simulink model "pfb_fir_1024c_32i_core"  (R2019a)
(part 4 of 32)

      |     set_param(gcb, 'MaskVisibilities',{'on','on','on','on','on'});
      | end
  pol1_in6_tap2 : Subsystem  AncestorBlock=casper_library_pfbs/tap_real  mask(pfb_tap_real){mult_latency=2, coeff_width=18, coeff_frac_width=17, delay=64, data_width=8, bram_latency=2, use_hdl=on, use_embedded=off}
      mask prompts: mult_latency "Multiplier Latency"; coeff_width "Coefficient Bit Width In"; coeff_frac_width "Coefficient Fractional Bits"; delay "Data/Sync Delay"; data_width "Data Bit Width In"; bram_latency "BRAM Latency"; use_hdl "Use behavioral HDL for multlipliers"; use_embedded "Use embedded multipliers"
      mask init: same as pfb_fir_1024c_32i_core/pfb_fir_real/pol1_in10_tap2
  pol1_in6_tap3 : Subsystem  AncestorBlock=casper_library_pfbs/tap_real  mask(pfb_tap_real){mult_latency=2, coeff_width=18, coeff_frac_width=17, delay=64, data_width=8, bram_latency=2, use_hdl=on, use_embedded=off}
      mask prompts: mult_latency "Multiplier Latency"; coeff_width "Coefficient Bit Width In"; coeff_frac_width "Coefficient Fractional Bits"; delay "Data/Sync Delay"; data_width "Data Bit Width In"; bram_latency "BRAM Latency"; use_hdl "Use behavioral HDL for multlipliers"; use_embedded "Use embedded multipliers"
      mask init: same as pfb_fir_1024c_32i_core/pfb_fir_real/pol1_in10_tap2
  pol1_in6_tap4 : Subsystem  AncestorBlock=casper_library_pfbs/tap_real  mask(pfb_tap_real){mult_latency=2, coeff_width=18, coeff_frac_width=17, delay=64, data_width=8, bram_latency=2, use_hdl=on, use_embedded=off}
      mask prompts: mult_latency "Multiplier Latency"; coeff_width "Coefficient Bit Width In"; coeff_frac_width "Coefficient Fractional Bits"; delay "Data/Sync Delay"; data_width "Data Bit Width In"; bram_latency "BRAM Latency"; use_hdl "Use behavioral HDL for multlipliers"; use_embedded "Use embedded multipliers"
      mask init: same as pfb_fir_1024c_32i_core/pfb_fir_real/pol1_in10_tap2
  pol1_in6_tap5 : Subsystem  AncestorBlock=casper_library_pfbs/tap_real  mask(pfb_tap_real){mult_latency=2, coeff_width=18, coeff_frac_width=17, delay=64, data_width=8, bram_latency=2, use_hdl=on, use_embedded=off}
      mask prompts: mult_latency "Multiplier Latency"; coeff_width "Coefficient Bit Width In"; coeff_frac_width "Coefficient Fractional Bits"; delay "Data/Sync Delay"; data_width "Data Bit Width In"; bram_latency "BRAM Latency"; use_hdl "Use behavioral HDL for multlipliers"; use_embedded "Use embedded multipliers"
      mask init: same as pfb_fir_1024c_32i_core/pfb_fir_real/pol1_in10_tap2
  pol1_in6_tap6 : Subsystem  AncestorBlock=casper_library_pfbs/tap_real  mask(pfb_tap_real){mult_latency=2, coeff_width=18, coeff_frac_width=17, delay=64, data_width=8, bram_latency=2, use_hdl=on, use_embedded=off}
      mask prompts: mult_latency "Multiplier Latency"; coeff_width "Coefficient Bit Width In"; coeff_frac_width "Coefficient Fractional Bits"; delay "Data/Sync Delay"; data_width "Data Bit Width In"; bram_latency "BRAM Latency"; use_hdl "Use behavioral HDL for multlipliers"; use_embedded "Use embedded multipliers"
      mask init: same as pfb_fir_1024c_32i_core/pfb_fir_real/pol1_in10_tap2
  pol1_in6_tap7 : Subsystem  AncestorBlock=casper_library_pfbs/tap_real  mask(pfb_tap_real){mult_latency=2, coeff_width=18, coeff_frac_width=17, delay=64, data_width=8, bram_latency=2, use_hdl=on, use_embedded=off}
      mask prompts: mult_latency "Multiplier Latency"; coeff_width "Coefficient Bit Width In"; coeff_frac_width "Coefficient Fractional Bits"; delay "Data/Sync Delay"; data_width "Data Bit Width In"; bram_latency "BRAM Latency"; use_hdl "Use behavioral HDL for multlipliers"; use_embedded "Use embedded multipliers"
      mask init: same as pfb_fir_1024c_32i_core/pfb_fir_real/pol1_in10_tap2
  pol1_in7_coeffs : Subsystem  AncestorBlock=casper_library_pfbs/pfb_coeff_gen  mask(pfb_coeff_gen){PFBSize=11, CoeffBitWidth=18, TotalTaps=8, CoeffDistMem=off, WindowType=hamming, bram_latency=2, n_inputs=5, nput=6, fwidth=1, debug_mode=off, fan_latency=1}
      mask prompts: PFBSize "Size of PFB: (2^? pnts)"; CoeffBitWidth "Bitwidth of Coefficients:"; TotalTaps "Total Number of Taps:"; CoeffDistMem "Implement Coeff Gen in Distributed Memory"; WindowType "Windowing Function:"; bram_latency "BRAM Latency"; n_inputs "Number of Simultaneous Inputs: (2^?)"; nput "This is input number:"; fwidth "Bin Width (normal=1)"; debug_mode "Debug mode - coeffs are a [1:pfb_size*taps] ramp."; fan_latency "Fanout latency"
      mask init: same as pfb_fir_1024c_32i_core/pfb_fir_real/pol1_in10_coeffs
      settings: AttributesFormatString=|
      | PFBSize=11, n_inputs=5,
      | taps=8, input=6
  pol1_in7_first_tap : Subsystem  AncestorBlock=casper_library_pfbs/first_tap_real  mask(first_tap_real){PFBSize=11, CoeffBitWidth=18, TotalTaps=8, BitWidthIn=8, WindowType=hamming, mult_latency=2, bram_latency=2, n_inputs=5, fwidth=1, use_hdl=on, use_embedded=off}
      mask prompts: PFBSize "Size of PFB: (2^? pnts)"; CoeffBitWidth "Bitwidth of Coefficients:"; TotalTaps "Total Number of Taps:"; BitWidthIn "Input Bitwidth:"; WindowType "Windowing Function:"; mult_latency "Mult Latency"; bram_latency "BRAM Latency"; n_inputs "Number of Simultaneous Inputs: (2^?)"; fwidth "Bit Width (normal=1)"; use_hdl "Use behavioral HDL for multlipliers"; use_embedded "Use embedded multipliers"
      mask init: same as pfb_fir_1024c_32i_core/pfb_fir_real/pol1_in10_first_tap
      settings: AttributesFormatString=taps=8
      mask TypeOptions WindowType: bartlett | barthannwin | blackman | blackmanharris | bohamwin | chebwin | flattopwin | gausswin | hamming | hann | kaiser | nuttallwin | parzenwin | rectwin | tukeywin | triang | userwindow
      mask Callback use_hdl:
      | use_hdl = get_param(gcb,'use_hdl');
      | if( strcmp(use_hdl,'on')),
      |     set_param(gcb, 'use_embedded','off');
      |     set_param(gcb, 'MaskVisibilities',{'on','on','on','on','on','on','on','on','on','on','off'});
      | else,
      |     set_param(gcb, 'MaskVisibilities',{'on','on','on','on','on','on','on','on','on','on','on'});
      | end
  pol1_in7_last_tap : Subsystem  AncestorBlock=casper_library_pfbs/last_tap_real  mask(last_tap_real){BitWidthIn=8, CoeffBitWidth=18, mult_latency=2, use_hdl=on, use_embedded=off}
      mask prompts: BitWidthIn "Input Bitwidth:"; CoeffBitWidth "Coeff Bitwidth:"; mult_latency "Mult Latency"; use_hdl "Use behavioral HDL for multlipliers"; use_embedded "Use embedded multipliers"
      mask init:
      | last_tap_real_init(gcb,...
      |     'BitWidthIn', BitWidthIn,...
      |     'CoeffBitWidth', CoeffBitWidth,...
      |     'mult_latency', mult_latency,...
      |     'use_hdl', use_hdl,...
      |     'use_embedded', use_embedded);
      mask Callback use_hdl:
      | use_hdl = get_param(gcb,'use_hdl');
      | if( strcmp(use_hdl,'on')),
      |     set_param(gcb, 'use_embedded','off');
      |     set_param(gcb, 'MaskVisibilities',{'on','on','on','on','off'});
      | else,
      |     set_param(gcb, 'MaskVisibilities',{'on','on','on','on','on'});
      | end
  pol1_in7_tap2 : Subsystem  AncestorBlock=casper_library_pfbs/tap_real  mask(pfb_tap_real){mult_latency=2, coeff_width=18, coeff_frac_width=17, delay=64, data_width=8, bram_latency=2, use_hdl=on, use_embedded=off}
      mask prompts: mult_latency "Multiplier Latency"; coeff_width "Coefficient Bit Width In"; coeff_frac_width "Coefficient Fractional Bits"; delay "Data/Sync Delay"; data_width "Data Bit Width In"; bram_latency "BRAM Latency"; use_hdl "Use behavioral HDL for multlipliers"; use_embedded "Use embedded multipliers"
      mask init: same as pfb_fir_1024c_32i_core/pfb_fir_real/pol1_in10_tap2
  pol1_in7_tap3 : Subsystem  AncestorBlock=casper_library_pfbs/tap_real  mask(pfb_tap_real){mult_latency=2, coeff_width=18, coeff_frac_width=17, delay=64, data_width=8, bram_latency=2, use_hdl=on, use_embedded=off}
      mask prompts: mult_latency "Multiplier Latency"; coeff_width "Coefficient Bit Width In"; coeff_frac_width "Coefficient Fractional Bits"; delay "Data/Sync Delay"; data_width "Data Bit Width In"; bram_latency "BRAM Latency"; use_hdl "Use behavioral HDL for multlipliers"; use_embedded "Use embedded multipliers"
      mask init: same as pfb_fir_1024c_32i_core/pfb_fir_real/pol1_in10_tap2
  pol1_in7_tap4 : Subsystem  AncestorBlock=casper_library_pfbs/tap_real  mask(pfb_tap_real){mult_latency=2, coeff_width=18, coeff_frac_width=17, delay=64, data_width=8, bram_latency=2, use_hdl=on, use_embedded=off}
      mask prompts: mult_latency "Multiplier Latency"; coeff_width "Coefficient Bit Width In"; coeff_frac_width "Coefficient Fractional Bits"; delay "Data/Sync Delay"; data_width "Data Bit Width In"; bram_latency "BRAM Latency"; use_hdl "Use behavioral HDL for multlipliers"; use_embedded "Use embedded multipliers"
      mask init: same as pfb_fir_1024c_32i_core/pfb_fir_real/pol1_in10_tap2
  pol1_in7_tap5 : Subsystem  AncestorBlock=casper_library_pfbs/tap_real  mask(pfb_tap_real){mult_latency=2, coeff_width=18, coeff_frac_width=17, delay=64, data_width=8, bram_latency=2, use_hdl=on, use_embedded=off}
      mask prompts: mult_latency "Multiplier Latency"; coeff_width "Coefficient Bit Width In"; coeff_frac_width "Coefficient Fractional Bits"; delay "Data/Sync Delay"; data_width "Data Bit Width In"; bram_latency "BRAM Latency"; use_hdl "Use behavioral HDL for multlipliers"; use_embedded "Use embedded multipliers"
      mask init: same as pfb_fir_1024c_32i_core/pfb_fir_real/pol1_in10_tap2
  pol1_in7_tap6 : Subsystem  AncestorBlock=casper_library_pfbs/tap_real  mask(pfb_tap_real){mult_latency=2, coeff_width=18, coeff_frac_width=17, delay=64, data_width=8, bram_latency=2, use_hdl=on, use_embedded=off}
      mask prompts: mult_latency "Multiplier Latency"; coeff_width "Coefficient Bit Width In"; coeff_frac_width "Coefficient Fractional Bits"; delay "Data/Sync Delay"; data_width "Data Bit Width In"; bram_latency "BRAM Latency"; use_hdl "Use behavioral HDL for multlipliers"; use_embedded "Use embedded multipliers"
      mask init: same as pfb_fir_1024c_32i_core/pfb_fir_real/pol1_in10_tap2
  pol1_in7_tap7 : Subsystem  AncestorBlock=casper_library_pfbs/tap_real  mask(pfb_tap_real){mult_latency=2, coeff_width=18, coeff_frac_width=17, delay=64, data_width=8, bram_latency=2, use_hdl=on, use_embedded=off}
      mask prompts: mult_latency "Multiplier Latency"; coeff_width "Coefficient Bit Width In"; coeff_frac_width "Coefficient Fractional Bits"; delay "Data/Sync Delay"; data_width "Data Bit Width In"; bram_latency "BRAM Latency"; use_hdl "Use behavioral HDL for multlipliers"; use_embedded "Use embedded multipliers"
      mask init: same as pfb_fir_1024c_32i_core/pfb_fir_real/pol1_in10_tap2
  pol1_in8_coeffs : Subsystem  AncestorBlock=casper_library_pfbs/pfb_coeff_gen  mask(pfb_coeff_gen){PFBSize=11, CoeffBitWidth=18, TotalTaps=8, CoeffDistMem=off, WindowType=hamming, bram_latency=2, n_inputs=5, nput=7, fwidth=1, debug_mode=off, fan_latency=1}
      mask prompts: PFBSize "Size of PFB: (2^? pnts)"; CoeffBitWidth "Bitwidth of Coefficients:"; TotalTaps "Total Number of Taps:"; CoeffDistMem "Implement Coeff Gen in Distributed Memory"; WindowType "Windowing Function:"; bram_latency "BRAM Latency"; n_inputs "Number of Simultaneous Inputs: (2^?)"; nput "This is input number:"; fwidth "Bin Width (normal=1)"; debug_mode "Debug mode - coeffs are a [1:pfb_size*taps] ramp."; fan_latency "Fanout latency"
      mask init: same as pfb_fir_1024c_32i_core/pfb_fir_real/pol1_in10_coeffs
      settings: AttributesFormatString=|
      | PFBSize=11, n_inputs=5,
      | taps=8, input=7
  pol1_in8_first_tap : Subsystem  AncestorBlock=casper_library_pfbs/first_tap_real  mask(first_tap_real){PFBSize=11, CoeffBitWidth=18, TotalTaps=8, BitWidthIn=8, WindowType=hamming, mult_latency=2, bram_latency=2, n_inputs=5, fwidth=1, use_hdl=on, use_embedded=off}
      mask prompts: PFBSize "Size of PFB: (2^? pnts)"; CoeffBitWidth "Bitwidth of Coefficients:"; TotalTaps "Total Number of Taps:"; BitWidthIn "Input Bitwidth:"; WindowType "Windowing Function:"; mult_latency "Mult Latency"; bram_latency "BRAM Latency"; n_inputs "Number of Simultaneous Inputs: (2^?)"; fwidth "Bit Width (normal=1)"; use_hdl "Use behavioral HDL for multlipliers"; use_embedded "Use embedded multipliers"
      mask init: same as pfb_fir_1024c_32i_core/pfb_fir_real/pol1_in10_first_tap
      settings: AttributesFormatString=taps=8
      mask TypeOptions WindowType: bartlett | barthannwin | blackman | blackmanharris | bohamwin | chebwin | flattopwin | gausswin | hamming | hann | kaiser | nuttallwin | parzenwin | rectwin | tukeywin | triang | userwindow
      mask Callback use_hdl:
      | use_hdl = get_param(gcb,'use_hdl');
      | if( strcmp(use_hdl,'on')),
      |     set_param(gcb, 'use_embedded','off');
      |     set_param(gcb, 'MaskVisibilities',{'on','on','on','on','on','on','on','on','on','on','off'});
      | else,
      |     set_param(gcb, 'MaskVisibilities',{'on','on','on','on','on','on','on','on','on','on','on'});
      | end
  pol1_in8_last_tap : Subsystem  AncestorBlock=casper_library_pfbs/last_tap_real  mask(last_tap_real){BitWidthIn=8, CoeffBitWidth=18, mult_latency=2, use_hdl=on, use_embedded=off}
      mask prompts: BitWidthIn "Input Bitwidth:"; CoeffBitWidth "Coeff Bitwidth:"; mult_latency "Mult Latency"; use_hdl "Use behavioral HDL for multlipliers"; use_embedded "Use embedded multipliers"
      mask init:
      | last_tap_real_init(gcb,...
      |     'BitWidthIn', BitWidthIn,...
      |     'CoeffBitWidth', CoeffBitWidth,...
      |     'mult_latency', mult_latency,...
      |     'use_hdl', use_hdl,...
      |     'use_embedded', use_embedded);
      mask Callback use_hdl:
      | use_hdl = get_param(gcb,'use_hdl');
      | if( strcmp(use_hdl,'on')),
      |     set_param(gcb, 'use_embedded','off');
      |     set_param(gcb, 'MaskVisibilities',{'on','on','on','on','off'});
      | else,
      |     set_param(gcb, 'MaskVisibilities',{'on','on','on','on','on'});
      | end
  pol1_in8_tap2 : Subsystem  AncestorBlock=casper_library_pfbs/tap_real  mask(pfb_tap_real){mult_latency=2, coeff_width=18, coeff_frac_width=17, delay=64, data_width=8, bram_latency=2, use_hdl=on, use_embedded=off}
      mask prompts: mult_latency "Multiplier Latency"; coeff_width "Coefficient Bit Width In"; coeff_frac_width "Coefficient Fractional Bits"; delay "Data/Sync Delay"; data_width "Data Bit Width In"; bram_latency "BRAM Latency"; use_hdl "Use behavioral HDL for multlipliers"; use_embedded "Use embedded multipliers"
      mask init: same as pfb_fir_1024c_32i_core/pfb_fir_real/pol1_in10_tap2
  pol1_in8_tap3 : Subsystem  AncestorBlock=casper_library_pfbs/tap_real  mask(pfb_tap_real){mult_latency=2, coeff_width=18, coeff_frac_width=17, delay=64, data_width=8, bram_latency=2, use_hdl=on, use_embedded=off}
      mask prompts: mult_latency "Multiplier Latency"; coeff_width "Coefficient Bit Width In"; coeff_frac_width "Coefficient Fractional Bits"; delay "Data/Sync Delay"; data_width "Data Bit Width In"; bram_latency "BRAM Latency"; use_hdl "Use behavioral HDL for multlipliers"; use_embedded "Use embedded multipliers"
      mask init: same as pfb_fir_1024c_32i_core/pfb_fir_real/pol1_in10_tap2
  pol1_in8_tap4 : Subsystem  AncestorBlock=casper_library_pfbs/tap_real  mask(pfb_tap_real){mult_latency=2, coeff_width=18, coeff_frac_width=17, delay=64, data_width=8, bram_latency=2, use_hdl=on, use_embedded=off}
      mask prompts: mult_latency "Multiplier Latency"; coeff_width "Coefficient Bit Width In"; coeff_frac_width "Coefficient Fractional Bits"; delay "Data/Sync Delay"; data_width "Data Bit Width In"; bram_latency "BRAM Latency"; use_hdl "Use behavioral HDL for multlipliers"; use_embedded "Use embedded multipliers"
      mask init: same as pfb_fir_1024c_32i_core/pfb_fir_real/pol1_in10_tap2
  pol1_in8_tap5 : Subsystem  AncestorBlock=casper_library_pfbs/tap_real  mask(pfb_tap_real){mult_latency=2, coeff_width=18, coeff_frac_width=17, delay=64, data_width=8, bram_latency=2, use_hdl=on, use_embedded=off}
      mask prompts: mult_latency "Multiplier Latency"; coeff_width "Coefficient Bit Width In"; coeff_frac_width "Coefficient Fractional Bits"; delay "Data/Sync Delay"; data_width "Data Bit Width In"; bram_latency "BRAM Latency"; use_hdl "Use behavioral HDL for multlipliers"; use_embedded "Use embedded multipliers"
      mask init: same as pfb_fir_1024c_32i_core/pfb_fir_real/pol1_in10_tap2
  pol1_in8_tap6 : Subsystem  AncestorBlock=casper_library_pfbs/tap_real  mask(pfb_tap_real){mult_latency=2, coeff_width=18, coeff_frac_width=17, delay=64, data_width=8, bram_latency=2, use_hdl=on, use_embedded=off}
      mask prompts: mult_latency "Multiplier Latency"; coeff_width "Coefficient Bit Width In"; coeff_frac_width "Coefficient Fractional Bits"; delay "Data/Sync Delay"; data_width "Data Bit Width In"; bram_latency "BRAM Latency"; use_hdl "Use behavioral HDL for multlipliers"; use_embedded "Use embedded multipliers"
      mask init: same as pfb_fir_1024c_32i_core/pfb_fir_real/pol1_in10_tap2
  pol1_in8_tap7 : Subsystem  AncestorBlock=casper_library_pfbs/tap_real  mask(pfb_tap_real){mult_latency=2, coeff_width=18, coeff_frac_width=17, delay=64, data_width=8, bram_latency=2, use_hdl=on, use_embedded=off}
      mask prompts: mult_latency "Multiplier Latency"; coeff_width "Coefficient Bit Width In"; coeff_frac_width "Coefficient Fractional Bits"; delay "Data/Sync Delay"; data_width "Data Bit Width In"; bram_latency "BRAM Latency"; use_hdl "Use behavioral HDL for multlipliers"; use_embedded "Use embedded multipliers"
      mask init: same as pfb_fir_1024c_32i_core/pfb_fir_real/pol1_in10_tap2
  pol1_in9_coeffs : Subsystem  AncestorBlock=casper_library_pfbs/pfb_coeff_gen  mask(pfb_coeff_gen){PFBSize=11, CoeffBitWidth=18, TotalTaps=8, CoeffDistMem=off, WindowType=hamming, bram_latency=2, n_inputs=5, nput=8, fwidth=1, debug_mode=off, fan_latency=1}
      mask prompts: PFBSize "Size of PFB: (2^? pnts)"; CoeffBitWidth "Bitwidth of Coefficients:"; TotalTaps "Total Number of Taps:"; CoeffDistMem "Implement Coeff Gen in Distributed Memory"; WindowType "Windowing Function:"; bram_latency "BRAM Latency"; n_inputs "Number of Simultaneous Inputs: (2^?)"; nput "This is input number:"; fwidth "Bin Width (normal=1)"; debug_mode "Debug mode - coeffs are a [1:pfb_size*taps] ramp."; fan_latency "Fanout latency"
      mask init: same as pfb_fir_1024c_32i_core/pfb_fir_real/pol1_in10_coeffs
      settings: AttributesFormatString=|
      | PFBSize=11, n_inputs=5,
      | taps=8, input=8
  pol1_in9_first_tap : Subsystem  AncestorBlock=casper_library_pfbs/first_tap_real  mask(first_tap_real){PFBSize=11, CoeffBitWidth=18, TotalTaps=8, BitWidthIn=8, WindowType=hamming, mult_latency=2, bram_latency=2, n_inputs=5, fwidth=1, use_hdl=on, use_embedded=off}
      mask prompts: PFBSize "Size of PFB: (2^? pnts)"; CoeffBitWidth "Bitwidth of Coefficients:"; TotalTaps "Total Number of Taps:"; BitWidthIn "Input Bitwidth:"; WindowType "Windowing Function:"; mult_latency "Mult Latency"; bram_latency "BRAM Latency"; n_inputs "Number of Simultaneous Inputs: (2^?)"; fwidth "Bit Width (normal=1)"; use_hdl "Use behavioral HDL for multlipliers"; use_embedded "Use embedded multipliers"
      mask init: same as pfb_fir_1024c_32i_core/pfb_fir_real/pol1_in10_first_tap
      settings: AttributesFormatString=taps=8
      mask TypeOptions WindowType: bartlett | barthannwin | blackman | blackmanharris | bohamwin | chebwin | flattopwin | gausswin | hamming | hann | kaiser | nuttallwin | parzenwin | rectwin | tukeywin | triang | userwindow
      mask Callback use_hdl:
      | use_hdl = get_param(gcb,'use_hdl');
      | if( strcmp(use_hdl,'on')),
      |     set_param(gcb, 'use_embedded','off');
      |     set_param(gcb, 'MaskVisibilities',{'on','on','on','on','on','on','on','on','on','on','off'});
      | else,
      |     set_param(gcb, 'MaskVisibilities',{'on','on','on','on','on','on','on','on','on','on','on'});
      | end
  pol1_in9_last_tap : Subsystem  AncestorBlock=casper_library_pfbs/last_tap_real  mask(last_tap_real){BitWidthIn=8, CoeffBitWidth=18, mult_latency=2, use_hdl=on, use_embedded=off}
      mask prompts: BitWidthIn "Input Bitwidth:"; CoeffBitWidth "Coeff Bitwidth:"; mult_latency "Mult Latency"; use_hdl "Use behavioral HDL for multlipliers"; use_embedded "Use embedded multipliers"
      mask init:
      | last_tap_real_init(gcb,...
      |     'BitWidthIn', BitWidthIn,...
      |     'CoeffBitWidth', CoeffBitWidth,...
      |     'mult_latency', mult_latency,...
      |     'use_hdl', use_hdl,...
      |     'use_embedded', use_embedded);
      mask Callback use_hdl:
      | use_hdl = get_param(gcb,'use_hdl');
      | if( strcmp(use_hdl,'on')),
      |     set_param(gcb, 'use_embedded','off');
      |     set_param(gcb, 'MaskVisibilities',{'on','on','on','on','off'});
      | else,
      |     set_param(gcb, 'MaskVisibilities',{'on','on','on','on','on'});
      | end
  pol1_in9_tap2 : Subsystem  AncestorBlock=casper_library_pfbs/tap_real  mask(pfb_tap_real){mult_latency=2, coeff_width=18, coeff_frac_width=17, delay=64, data_width=8, bram_latency=2, use_hdl=on, use_embedded=off}
      mask prompts: mult_latency "Multiplier Latency"; coeff_width "Coefficient Bit Width In"; coeff_frac_width "Coefficient Fractional Bits"; delay "Data/Sync Delay"; data_width "Data Bit Width In"; bram_latency "BRAM Latency"; use_hdl "Use behavioral HDL for multlipliers"; use_embedded "Use embedded multipliers"
      mask init: same as pfb_fir_1024c_32i_core/pfb_fir_real/pol1_in10_tap2
  pol1_in9_tap3 : Subsystem  AncestorBlock=casper_library_pfbs/tap_real  mask(pfb_tap_real){mult_latency=2, coeff_width=18, coeff_frac_width=17, delay=64, data_width=8, bram_latency=2, use_hdl=on, use_embedded=off}
      mask prompts: mult_latency "Multiplier Latency"; coeff_width "Coefficient Bit Width In"; coeff_frac_width "Coefficient Fractional Bits"; delay "Data/Sync Delay"; data_width "Data Bit Width In"; bram_latency "BRAM Latency"; use_hdl "Use behavioral HDL for multlipliers"; use_embedded "Use embedded multipliers"
      mask init: same as pfb_fir_1024c_32i_core/pfb_fir_real/pol1_in10_tap2
  pol1_in9_tap4 : Subsystem  AncestorBlock=casper_library_pfbs/tap_real  mask(pfb_tap_real){mult_latency=2, coeff_width=18, coeff_frac_width=17, delay=64, data_width=8, bram_latency=2, use_hdl=on, use_embedded=off}
      mask prompts: mult_latency "Multiplier Latency"; coeff_width "Coefficient Bit Width In"; coeff_frac_width "Coefficient Fractional Bits"; delay "Data/Sync Delay"; data_width "Data Bit Width In"; bram_latency "BRAM Latency"; use_hdl "Use behavioral HDL for multlipliers"; use_embedded "Use embedded multipliers"
      mask init: same as pfb_fir_1024c_32i_core/pfb_fir_real/pol1_in10_tap2
  pol1_in9_tap5 : Subsystem  AncestorBlock=casper_library_pfbs/tap_real  mask(pfb_tap_real){mult_latency=2, coeff_width=18, coeff_frac_width=17, delay=64, data_width=8, bram_latency=2, use_hdl=on, use_embedded=off}
      mask prompts: mult_latency "Multiplier Latency"; coeff_width "Coefficient Bit Width In"; coeff_frac_width "Coefficient Fractional Bits"; delay "Data/Sync Delay"; data_width "Data Bit Width In"; bram_latency "BRAM Latency"; use_hdl "Use behavioral HDL for multlipliers"; use_embedded "Use embedded multipliers"
      mask init: same as pfb_fir_1024c_32i_core/pfb_fir_real/pol1_in10_tap2
  pol1_in9_tap6 : Subsystem  AncestorBlock=casper_library_pfbs/tap_real  mask(pfb_tap_real){mult_latency=2, coeff_width=18, coeff_frac_width=17, delay=64, data_width=8, bram_latency=2, use_hdl=on, use_embedded=off}
      mask prompts: mult_latency "Multiplier Latency"; coeff_width "Coefficient Bit Width In"; coeff_frac_width "Coefficient Fractional Bits"; delay "Data/Sync Delay"; data_width "Data Bit Width In"; bram_latency "BRAM Latency"; use_hdl "Use behavioral HDL for multlipliers"; use_embedded "Use embedded multipliers"
      mask init: same as pfb_fir_1024c_32i_core/pfb_fir_real/pol1_in10_tap2
  pol1_in9_tap7 : Subsystem  AncestorBlock=casper_library_pfbs/tap_real  mask(pfb_tap_real){mult_latency=2, coeff_width=18, coeff_frac_width=17, delay=64, data_width=8, bram_latency=2, use_hdl=on, use_embedded=off}
      mask prompts: mult_latency "Multiplier Latency"; coeff_width "Coefficient Bit Width In"; coeff_frac_width "Coefficient Fractional Bits"; delay "Data/Sync Delay"; data_width "Data Bit Width In"; bram_latency "BRAM Latency"; use_hdl "Use behavioral HDL for multlipliers"; use_embedded "Use embedded multipliers"
      mask init: same as pfb_fir_1024c_32i_core/pfb_fir_real/pol1_in10_tap2
  scale_1_{1..32} (32 alike) : xbsIndex_r4/Scale  scale_factor=-1  dbl_ovrd=off  block_type=scale
  sync_out : Outport
  pol1_out1 : Outport  Port=2
  pol1_out2 : Outport  Port=3
  pol1_out3 : Outport  Port=4
  pol1_out4 : Outport  Port=5
  pol1_out5 : Outport  Port=6
  pol1_out6 : Outport  Port=7
  pol1_out7 : Outport  Port=8
  pol1_out8 : Outport  Port=9
  pol1_out9 : Outport  Port=10
  pol1_out10 : Outport  Port=11
  pol1_out11 : Outport  Port=12
  pol1_out12 : Outport  Port=13
  pol1_out13 : Outport  Port=14
  pol1_out14 : Outport  Port=15
  pol1_out15 : Outport  Port=16
  pol1_out16 : Outport  Port=17
  pol1_out17 : Outport  Port=18
  pol1_out18 : Outport  Port=19
  pol1_out19 : Outport  Port=20
  pol1_out20 : Outport  Port=21
  pol1_out21 : Outport  Port=22
  pol1_out22 : Outport  Port=23
  pol1_out23 : Outport  Port=24
  pol1_out24 : Outport  Port=25
  pol1_out25 : Outport  Port=26
  pol1_out26 : Outport  Port=27
  pol1_out27 : Outport  Port=28
  pol1_out28 : Outport  Port=29
  pol1_out29 : Outport  Port=30
  pol1_out30 : Outport  Port=31
  pol1_out31 : Outport  Port=32
  pol1_out32 : Outport  Port=33
  wires:
  pol1_in1/1 -> pol1_in1_coeffs/1(din)
  sync/1 -> pol1_in1_coeffs/2(sync), pol1_in2_coeffs/2(sync), pol1_in3_coeffs/2(sync), pol1_in4_coeffs/2(sync), pol1_in5_coeffs/2(sync), pol1_in6_coeffs/2(sync), pol1_in7_coeffs/2(sync), pol1_in8_coeffs/2(sync), pol1_in9_coeffs/2(sync), pol1_in10_coeffs/2(sync), pol1_in11_coeffs/2(sync), pol1_in12_coeffs/2(sync), pol1_in13_coeffs/2(sync), pol1_in14_coeffs/2(sync), pol1_in15_coeffs/2(sync), pol1_in16_coeffs/2(sync), pol1_in17_coeffs/2(sync), pol1_in18_coeffs/2(sync), pol1_in19_coeffs/2(sync), pol1_in20_coeffs/2(sync), pol1_in21_coeffs/2(sync), pol1_in22_coeffs/2(sync), pol1_in23_coeffs/2(sync), pol1_in24_coeffs/2(sync), pol1_in25_coeffs/2(sync), pol1_in26_coeffs/2(sync), pol1_in27_coeffs/2(sync), pol1_in28_coeffs/2(sync), pol1_in29_coeffs/2(sync), pol1_in30_coeffs/2(sync), pol1_in31_coeffs/2(sync), pol1_in32_coeffs/2(sync)
  pol1_in1_coeffs/1(dout) -> pol1_in1_first_tap/1(din)
  pol1_in1_coeffs/2(sync_out) -> pol1_in1_first_tap/2(sync), pol1_in2_first_tap/2(sync), pol1_in3_first_tap/2(sync), pol1_in4_first_tap/2(sync), pol1_in5_first_tap/2(sync), pol1_in6_first_tap/2(sync), pol1_in7_first_tap/2(sync), pol1_in8_first_tap/2(sync), pol1_in9_first_tap/2(sync), pol1_in10_first_tap/2(sync), pol1_in11_first_tap/2(sync), pol1_in12_first_tap/2(sync), pol1_in13_first_tap/2(sync), pol1_in14_first_tap/2(sync), pol1_in15_first_tap/2(sync), pol1_in16_first_tap/2(sync), pol1_in17_first_tap/2(sync), pol1_in18_first_tap/2(sync), pol1_in19_first_tap/2(sync), pol1_in20_first_tap/2(sync), pol1_in21_first_tap/2(sync), pol1_in22_first_tap/2(sync), pol1_in23_first_tap/2(sync), pol1_in24_first_tap/2(sync), pol1_in25_first_tap/2(sync), pol1_in26_first_tap/2(sync), pol1_in27_first_tap/2(sync), pol1_in28_first_tap/2(sync), pol1_in29_first_tap/2(sync), pol1_in30_first_tap/2(sync), pol1_in31_first_tap/2(sync), pol1_in32_first_tap/2(sync)
  pol1_in1_coeffs/3(coeff) -> pol1_in1_first_tap/3(coeffs)
  pol1_in2/1 -> pol1_in2_coeffs/1(din)
  pol1_in2_coeffs/1(dout) -> pol1_in2_first_tap/1(din)
  pol1_in2_coeffs/3(coeff) -> pol1_in2_first_tap/3(coeffs)
  pol1_in3/1 -> pol1_in3_coeffs/1(din)
  pol1_in3_coeffs/1(dout) -> pol1_in3_first_tap/1(din)
  pol1_in3_coeffs/3(coeff) -> pol1_in3_first_tap/3(coeffs)
  pol1_in4/1 -> pol1_in4_coeffs/1(din)
  pol1_in4_coeffs/1(dout) -> pol1_in4_first_tap/1(din)
  pol1_in4_coeffs/3(coeff) -> pol1_in4_first_tap/3(coeffs)
  pol1_in5/1 -> pol1_in5_coeffs/1(din)
  pol1_in5_coeffs/1(dout) -> pol1_in5_first_tap/1(din)
  pol1_in5_coeffs/3(coeff) -> pol1_in5_first_tap/3(coeffs)
  pol1_in6/1 -> pol1_in6_coeffs/1(din)
  pol1_in6_coeffs/1(dout) -> pol1_in6_first_tap/1(din)
  pol1_in6_coeffs/3(coeff) -> pol1_in6_first_tap/3(coeffs)
  pol1_in7/1 -> pol1_in7_coeffs/1(din)
  pol1_in7_coeffs/1(dout) -> pol1_in7_first_tap/1(din)
  pol1_in7_coeffs/3(coeff) -> pol1_in7_first_tap/3(coeffs)
  pol1_in8/1 -> pol1_in8_coeffs/1(din)
  pol1_in8_coeffs/1(dout) -> pol1_in8_first_tap/1(din)
  pol1_in8_coeffs/3(coeff) -> pol1_in8_first_tap/3(coeffs)
  pol1_in9/1 -> pol1_in9_coeffs/1(din)
  pol1_in9_coeffs/1(dout) -> pol1_in9_first_tap/1(din)
  pol1_in9_coeffs/3(coeff) -> pol1_in9_first_tap/3(coeffs)
  pol1_in10/1 -> pol1_in10_coeffs/1(din)
  pol1_in10_coeffs/1(dout) -> pol1_in10_first_tap/1(din)
  pol1_in10_coeffs/3(coeff) -> pol1_in10_first_tap/3(coeffs)
  pol1_in11/1 -> pol1_in11_coeffs/1(din)
  pol1_in11_coeffs/1(dout) -> pol1_in11_first_tap/1(din)
  pol1_in11_coeffs/3(coeff) -> pol1_in11_first_tap/3(coeffs)
  pol1_in12/1 -> pol1_in12_coeffs/1(din)
  pol1_in12_coeffs/1(dout) -> pol1_in12_first_tap/1(din)
  pol1_in12_coeffs/3(coeff) -> pol1_in12_first_tap/3(coeffs)
  pol1_in13/1 -> pol1_in13_coeffs/1(din)
  pol1_in13_coeffs/1(dout) -> pol1_in13_first_tap/1(din)
  pol1_in13_coeffs/3(coeff) -> pol1_in13_first_tap/3(coeffs)
  pol1_in14/1 -> pol1_in14_coeffs/1(din)
  pol1_in14_coeffs/1(dout) -> pol1_in14_first_tap/1(din)
  pol1_in14_coeffs/3(coeff) -> pol1_in14_first_tap/3(coeffs)
  pol1_in15/1 -> pol1_in15_coeffs/1(din)
  pol1_in15_coeffs/1(dout) -> pol1_in15_first_tap/1(din)
  pol1_in15_coeffs/3(coeff) -> pol1_in15_first_tap/3(coeffs)
  pol1_in16/1 -> pol1_in16_coeffs/1(din)
  pol1_in16_coeffs/1(dout) -> pol1_in16_first_tap/1(din)
  pol1_in16_coeffs/3(coeff) -> pol1_in16_first_tap/3(coeffs)
  pol1_in17/1 -> pol1_in17_coeffs/1(din)
  pol1_in17_coeffs/1(dout) -> pol1_in17_first_tap/1(din)
  pol1_in17_coeffs/3(coeff) -> pol1_in17_first_tap/3(coeffs)
  pol1_in18/1 -> pol1_in18_coeffs/1(din)
  pol1_in18_coeffs/1(dout) -> pol1_in18_first_tap/1(din)
  pol1_in18_coeffs/3(coeff) -> pol1_in18_first_tap/3(coeffs)
  pol1_in19/1 -> pol1_in19_coeffs/1(din)
  pol1_in19_coeffs/1(dout) -> pol1_in19_first_tap/1(din)
  pol1_in19_coeffs/3(coeff) -> pol1_in19_first_tap/3(coeffs)
  pol1_in20/1 -> pol1_in20_coeffs/1(din)
  pol1_in20_coeffs/1(dout) -> pol1_in20_first_tap/1(din)
  pol1_in20_coeffs/3(coeff) -> pol1_in20_first_tap/3(coeffs)
  pol1_in21/1 -> pol1_in21_coeffs/1(din)
  pol1_in21_coeffs/1(dout) -> pol1_in21_first_tap/1(din)
  pol1_in21_coeffs/3(coeff) -> pol1_in21_first_tap/3(coeffs)
  pol1_in22/1 -> pol1_in22_coeffs/1(din)
  pol1_in22_coeffs/1(dout) -> pol1_in22_first_tap/1(din)
  pol1_in22_coeffs/3(coeff) -> pol1_in22_first_tap/3(coeffs)
  pol1_in23/1 -> pol1_in23_coeffs/1(din)
  pol1_in23_coeffs/1(dout) -> pol1_in23_first_tap/1(din)
  pol1_in23_coeffs/3(coeff) -> pol1_in23_first_tap/3(coeffs)
  pol1_in24/1 -> pol1_in24_coeffs/1(din)
  pol1_in24_coeffs/1(dout) -> pol1_in24_first_tap/1(din)
  pol1_in24_coeffs/3(coeff) -> pol1_in24_first_tap/3(coeffs)
  pol1_in25/1 -> pol1_in25_coeffs/1(din)
  pol1_in25_coeffs/1(dout) -> pol1_in25_first_tap/1(din)
  pol1_in25_coeffs/3(coeff) -> pol1_in25_first_tap/3(coeffs)
  pol1_in26/1 -> pol1_in26_coeffs/1(din)
  pol1_in26_coeffs/1(dout) -> pol1_in26_first_tap/1(din)
  pol1_in26_coeffs/3(coeff) -> pol1_in26_first_tap/3(coeffs)
  pol1_in27/1 -> pol1_in27_coeffs/1(din)
  pol1_in27_coeffs/1(dout) -> pol1_in27_first_tap/1(din)
  pol1_in27_coeffs/3(coeff) -> pol1_in27_first_tap/3(coeffs)
  pol1_in28/1 -> pol1_in28_coeffs/1(din)
  pol1_in28_coeffs/1(dout) -> pol1_in28_first_tap/1(din)
  pol1_in28_coeffs/3(coeff) -> pol1_in28_first_tap/3(coeffs)
  pol1_in29/1 -> pol1_in29_coeffs/1(din)
  pol1_in29_coeffs/1(dout) -> pol1_in29_first_tap/1(din)
  pol1_in29_coeffs/3(coeff) -> pol1_in29_first_tap/3(coeffs)
  pol1_in30/1 -> pol1_in30_coeffs/1(din)
  pol1_in30_coeffs/1(dout) -> pol1_in30_first_tap/1(din)
  pol1_in30_coeffs/3(coeff) -> pol1_in30_first_tap/3(coeffs)
  pol1_in31/1 -> pol1_in31_coeffs/1(din)
  pol1_in31_coeffs/1(dout) -> pol1_in31_first_tap/1(din)
  pol1_in31_coeffs/3(coeff) -> pol1_in31_first_tap/3(coeffs)
  pol1_in32/1 -> pol1_in32_coeffs/1(din)
  pol1_in32_coeffs/1(dout) -> pol1_in32_first_tap/1(din)
  pol1_in32_coeffs/3(coeff) -> pol1_in32_first_tap/3(coeffs)
  adder_1_1/1(sync_out) -> delay1/1
  delay1/1 -> sync_out/1
  adder_1_1/2(dout) -> scale_1_1/1
  scale_1_1/1 -> convert_1_1/1
  convert_1_1/1 -> pol1_out1/1
  adder_1_2/2(dout) -> scale_1_2/1
  scale_1_2/1 -> convert_1_2/1
  convert_1_2/1 -> pol1_out2/1
  adder_1_3/2(dout) -> scale_1_3/1
  scale_1_3/1 -> convert_1_3/1
  convert_1_3/1 -> pol1_out3/1
  adder_1_4/2(dout) -> scale_1_4/1
  scale_1_4/1 -> convert_1_4/1
  convert_1_4/1 -> pol1_out4/1
  adder_1_5/2(dout) -> scale_1_5/1
  scale_1_5/1 -> convert_1_5/1
  convert_1_5/1 -> pol1_out5/1
  adder_1_6/2(dout) -> scale_1_6/1
  scale_1_6/1 -> convert_1_6/1
  convert_1_6/1 -> pol1_out6/1
  adder_1_7/2(dout) -> scale_1_7/1
  scale_1_7/1 -> convert_1_7/1
  convert_1_7/1 -> pol1_out7/1
  adder_1_8/2(dout) -> scale_1_8/1
  scale_1_8/1 -> convert_1_8/1
  convert_1_8/1 -> pol1_out8/1
  adder_1_9/2(dout) -> scale_1_9/1
  scale_1_9/1 -> convert_1_9/1
  convert_1_9/1 -> pol1_out9/1
  adder_1_10/2(dout) -> scale_1_10/1
  scale_1_10/1 -> convert_1_10/1
  convert_1_10/1 -> pol1_out10/1
  adder_1_11/2(dout) -> scale_1_11/1
  scale_1_11/1 -> convert_1_11/1
  convert_1_11/1 -> pol1_out11/1
  adder_1_12/2(dout) -> scale_1_12/1
  scale_1_12/1 -> convert_1_12/1
  convert_1_12/1 -> pol1_out12/1
  adder_1_13/2(dout) -> scale_1_13/1
  scale_1_13/1 -> convert_1_13/1
  convert_1_13/1 -> pol1_out13/1
  adder_1_14/2(dout) -> scale_1_14/1
  scale_1_14/1 -> convert_1_14/1
  convert_1_14/1 -> pol1_out14/1
  adder_1_15/2(dout) -> scale_1_15/1
  scale_1_15/1 -> convert_1_15/1
  convert_1_15/1 -> pol1_out15/1
  adder_1_16/2(dout) -> scale_1_16/1
  scale_1_16/1 -> convert_1_16/1
  convert_1_16/1 -> pol1_out16/1
  adder_1_17/2(dout) -> scale_1_17/1
  scale_1_17/1 -> convert_1_17/1
  convert_1_17/1 -> pol1_out17/1
  adder_1_18/2(dout) -> scale_1_18/1
  scale_1_18/1 -> convert_1_18/1
  convert_1_18/1 -> pol1_out18/1
  adder_1_19/2(dout) -> scale_1_19/1
  scale_1_19/1 -> convert_1_19/1
  convert_1_19/1 -> pol1_out19/1
  adder_1_20/2(dout) -> scale_1_20/1
  scale_1_20/1 -> convert_1_20/1
  convert_1_20/1 -> pol1_out20/1
  adder_1_21/2(dout) -> scale_1_21/1
  scale_1_21/1 -> convert_1_21/1
  convert_1_21/1 -> pol1_out21/1
  adder_1_22/2(dout) -> scale_1_22/1
  scale_1_22/1 -> convert_1_22/1
  convert_1_22/1 -> pol1_out22/1
  adder_1_23/2(dout) -> scale_1_23/1
  scale_1_23/1 -> convert_1_23/1
  convert_1_23/1 -> pol1_out23/1
  adder_1_24/2(dout) -> scale_1_24/1
  scale_1_24/1 -> convert_1_24/1
  convert_1_24/1 -> pol1_out24/1
  adder_1_25/2(dout) -> scale_1_25/1
  scale_1_25/1 -> convert_1_25/1
  convert_1_25/1 -> pol1_out25/1
  adder_1_26/2(dout) -> scale_1_26/1
  scale_1_26/1 -> convert_1_26/1
  convert_1_26/1 -> pol1_out26/1
  adder_1_27/2(dout) -> scale_1_27/1
  scale_1_27/1 -> convert_1_27/1
  convert_1_27/1 -> pol1_out27/1
  adder_1_28/2(dout) -> scale_1_28/1
  scale_1_28/1 -> convert_1_28/1
  convert_1_28/1 -> pol1_out28/1
  adder_1_29/2(dout) -> scale_1_29/1
  scale_1_29/1 -> convert_1_29/1
  convert_1_29/1 -> pol1_out29/1
  adder_1_30/2(dout) -> scale_1_30/1
  scale_1_30/1 -> convert_1_30/1
  convert_1_30/1 -> pol1_out30/1
  adder_1_31/2(dout) -> scale_1_31/1
  scale_1_31/1 -> convert_1_31/1
  convert_1_31/1 -> pol1_out31/1
  adder_1_32/2(dout) -> scale_1_32/1
  scale_1_32/1 -> convert_1_32/1
  convert_1_32/1 -> pol1_out32/1
  pol1_in1_first_tap/1(dout) -> pol1_in1_tap2/1(din)
  pol1_in1_first_tap/2(sync_out) -> pol1_in1_tap2/2(sync)
  pol1_in1_first_tap/3(coeff_out) -> pol1_in1_tap2/3(coeff)
  pol1_in1_first_tap/4(taps_out) -> adder_1_1/2(din1)
  pol1_in1_tap2/1(dout) -> pol1_in1_tap3/1(din)
  pol1_in1_tap2/2(sync_out) -> pol1_in1_tap3/2(sync)
  pol1_in1_tap2/3(coeff_out) -> pol1_in1_tap3/3(coeff)
  pol1_in1_tap2/4(taps_out) -> adder_1_1/3(din2)
  pol1_in1_tap3/1(dout) -> pol1_in1_tap4/1(din)
  pol1_in1_tap3/2(sync_out) -> pol1_in1_tap4/2(sync)
  pol1_in1_tap3/3(coeff_out) -> pol1_in1_tap4/3(coeff)
  pol1_in1_tap3/4(taps_out) -> adder_1_1/4(din3)
  pol1_in1_tap4/1(dout) -> pol1_in1_tap5/1(din)
  pol1_in1_tap4/2(sync_out) -> pol1_in1_tap5/2(sync)
  pol1_in1_tap4/3(coeff_out) -> pol1_in1_tap5/3(coeff)
  pol1_in1_tap4/4(taps_out) -> adder_1_1/5(din4)
  pol1_in1_tap5/1(dout) -> pol1_in1_tap6/1(din)
  pol1_in1_tap5/2(sync_out) -> pol1_in1_tap6/2(sync)
  pol1_in1_tap5/3(coeff_out) -> pol1_in1_tap6/3(coeff)
  pol1_in1_tap5/4(taps_out) -> adder_1_1/6(din5)
  pol1_in1_tap6/1(dout) -> pol1_in1_tap7/1(din)
  pol1_in1_tap6/2(sync_out) -> pol1_in1_tap7/2(sync)
  pol1_in1_tap6/3(coeff_out) -> pol1_in1_tap7/3(coeff)
  pol1_in1_tap6/4(taps_out) -> adder_1_1/7(din6)
  pol1_in1_last_tap/2(sync_out) -> adder_1_1/1(sync)
  pol1_in1_last_tap/1(tap_out) -> adder_1_1/9(din8)
  pol1_in1_tap7/1(dout) -> pol1_in1_last_tap/1(din)
  pol1_in1_tap7/2(sync_out) -> pol1_in1_last_tap/2(sync)
  pol1_in1_tap7/3(coeff_out) -> pol1_in1_last_tap/3(coeff)
  pol1_in1_tap7/4(taps_out) -> adder_1_1/8(din7)
  pol1_in2_first_tap/1(dout) -> pol1_in2_tap2/1(din)
  pol1_in2_first_tap/2(sync_out) -> pol1_in2_tap2/2(sync)
  pol1_in2_first_tap/3(coeff_out) -> pol1_in2_tap2/3(coeff)
  pol1_in2_first_tap/4(taps_out) -> adder_1_2/2(din1)
  pol1_in2_tap2/1(dout) -> pol1_in2_tap3/1(din)
  pol1_in2_tap2/2(sync_out) -> pol1_in2_tap3/2(sync)
  pol1_in2_tap2/3(coeff_out) -> pol1_in2_tap3/3(coeff)
  pol1_in2_tap2/4(taps_out) -> adder_1_2/3(din2)
  pol1_in2_tap3/1(dout) -> pol1_in2_tap4/1(din)
  pol1_in2_tap3/2(sync_out) -> pol1_in2_tap4/2(sync)
  pol1_in2_tap3/3(coeff_out) -> pol1_in2_tap4/3(coeff)
  pol1_in2_tap3/4(taps_out) -> adder_1_2/4(din3)
  pol1_in2_tap4/1(dout) -> pol1_in2_tap5/1(din)
  pol1_in2_tap4/2(sync_out) -> pol1_in2_tap5/2(sync)
  pol1_in2_tap4/3(coeff_out) -> pol1_in2_tap5/3(coeff)
  pol1_in2_tap4/4(taps_out) -> adder_1_2/5(din4)
  pol1_in2_tap5/1(dout) -> pol1_in2_tap6/1(din)
  pol1_in2_tap5/2(sync_out) -> pol1_in2_tap6/2(sync)
  pol1_in2_tap5/3(coeff_out) -> pol1_in2_tap6/3(coeff)
  pol1_in2_tap5/4(taps_out) -> adder_1_2/6(din5)
  pol1_in2_tap6/1(dout) -> pol1_in2_tap7/1(din)
  pol1_in2_tap6/2(sync_out) -> pol1_in2_tap7/2(sync)
  pol1_in2_tap6/3(coeff_out) -> pol1_in2_tap7/3(coeff)
  pol1_in2_tap6/4(taps_out) -> adder_1_2/7(din6)
  pol1_in2_last_tap/2(sync_out) -> adder_1_2/1(sync)
  pol1_in2_last_tap/1(tap_out) -> adder_1_2/9(din8)
  pol1_in2_tap7/1(dout) -> pol1_in2_last_tap/1(din)
  pol1_in2_tap7/2(sync_out) -> pol1_in2_last_tap/2(sync)
  pol1_in2_tap7/3(coeff_out) -> pol1_in2_last_tap/3(coeff)
  pol1_in2_tap7/4(taps_out) -> adder_1_2/8(din7)
  pol1_in3_first_tap/1(dout) -> pol1_in3_tap2/1(din)
  pol1_in3_first_tap/2(sync_out) -> pol1_in3_tap2/2(sync)
  pol1_in3_first_tap/3(coeff_out) -> pol1_in3_tap2/3(coeff)
  pol1_in3_first_tap/4(taps_out) -> adder_1_3/2(din1)
  pol1_in3_tap2/1(dout) -> pol1_in3_tap3/1(din)
  pol1_in3_tap2/2(sync_out) -> pol1_in3_tap3/2(sync)
  pol1_in3_tap2/3(coeff_out) -> pol1_in3_tap3/3(coeff)
  pol1_in3_tap2/4(taps_out) -> adder_1_3/3(din2)
  pol1_in3_tap3/1(dout) -> pol1_in3_tap4/1(din)
  pol1_in3_tap3/2(sync_out) -> pol1_in3_tap4/2(sync)
  pol1_in3_tap3/3(coeff_out) -> pol1_in3_tap4/3(coeff)
  pol1_in3_tap3/4(taps_out) -> adder_1_3/4(din3)
  pol1_in3_tap4/1(dout) -> pol1_in3_tap5/1(din)
  pol1_in3_tap4/2(sync_out) -> pol1_in3_tap5/2(sync)
  pol1_in3_tap4/3(coeff_out) -> pol1_in3_tap5/3(coeff)
  pol1_in3_tap4/4(taps_out) -> adder_1_3/5(din4)
  pol1_in3_tap5/1(dout) -> pol1_in3_tap6/1(din)
  pol1_in3_tap5/2(sync_out) -> pol1_in3_tap6/2(sync)
  pol1_in3_tap5/3(coeff_out) -> pol1_in3_tap6/3(coeff)
  pol1_in3_tap5/4(taps_out) -> adder_1_3/6(din5)
  pol1_in3_tap6/1(dout) -> pol1_in3_tap7/1(din)
  pol1_in3_tap6/2(sync_out) -> pol1_in3_tap7/2(sync)
  pol1_in3_tap6/3(coeff_out) -> pol1_in3_tap7/3(coeff)
  pol1_in3_tap6/4(taps_out) -> adder_1_3/7(din6)
  pol1_in3_last_tap/2(sync_out) -> adder_1_3/1(sync)
  pol1_in3_last_tap/1(tap_out) -> adder_1_3/9(din8)
  pol1_in3_tap7/1(dout) -> pol1_in3_last_tap/1(din)
  pol1_in3_tap7/2(sync_out) -> pol1_in3_last_tap/2(sync)
  pol1_in3_tap7/3(coeff_out) -> pol1_in3_last_tap/3(coeff)
  pol1_in3_tap7/4(taps_out) -> adder_1_3/8(din7)
  pol1_in4_first_tap/1(dout) -> pol1_in4_tap2/1(din)
  pol1_in4_first_tap/2(sync_out) -> pol1_in4_tap2/2(sync)
  pol1_in4_first_tap/3(coeff_out) -> pol1_in4_tap2/3(coeff)
  pol1_in4_first_tap/4(taps_out) -> adder_1_4/2(din1)
  pol1_in4_tap2/1(dout) -> pol1_in4_tap3/1(din)
  pol1_in4_tap2/2(sync_out) -> pol1_in4_tap3/2(sync)
  pol1_in4_tap2/3(coeff_out) -> pol1_in4_tap3/3(coeff)
  pol1_in4_tap2/4(taps_out) -> adder_1_4/3(din2)
  pol1_in4_tap3/1(dout) -> pol1_in4_tap4/1(din)
  pol1_in4_tap3/2(sync_out) -> pol1_in4_tap4/2(sync)
  pol1_in4_tap3/3(coeff_out) -> pol1_in4_tap4/3(coeff)
  pol1_in4_tap3/4(taps_out) -> adder_1_4/4(din3)
  pol1_in4_tap4/1(dout) -> pol1_in4_tap5/1(din)
  pol1_in4_tap4/2(sync_out) -> pol1_in4_tap5/2(sync)
  pol1_in4_tap4/3(coeff_out) -> pol1_in4_tap5/3(coeff)
  pol1_in4_tap4/4(taps_out) -> adder_1_4/5(din4)
  pol1_in4_tap5/1(dout) -> pol1_in4_tap6/1(din)
  pol1_in4_tap5/2(sync_out) -> pol1_in4_tap6/2(sync)
  pol1_in4_tap5/3(coeff_out) -> pol1_in4_tap6/3(coeff)
  pol1_in4_tap5/4(taps_out) -> adder_1_4/6(din5)
  pol1_in4_tap6/1(dout) -> pol1_in4_tap7/1(din)
  pol1_in4_tap6/2(sync_out) -> pol1_in4_tap7/2(sync)
  pol1_in4_tap6/3(coeff_out) -> pol1_in4_tap7/3(coeff)
  pol1_in4_tap6/4(taps_out) -> adder_1_4/7(din6)
  pol1_in4_last_tap/2(sync_out) -> adder_1_4/1(sync)
  pol1_in4_last_tap/1(tap_out) -> adder_1_4/9(din8)
  pol1_in4_tap7/1(dout) -> pol1_in4_last_tap/1(din)
  pol1_in4_tap7/2(sync_out) -> pol1_in4_last_tap/2(sync)
  pol1_in4_tap7/3(coeff_out) -> pol1_in4_last_tap/3(coeff)
  pol1_in4_tap7/4(taps_out) -> adder_1_4/8(din7)
  pol1_in5_first_tap/1(dout) -> pol1_in5_tap2/1(din)
  pol1_in5_first_tap/2(sync_out) -> pol1_in5_tap2/2(sync)
  pol1_in5_first_tap/3(coeff_out) -> pol1_in5_tap2/3(coeff)
  pol1_in5_first_tap/4(taps_out) -> adder_1_5/2(din1)
  pol1_in5_tap2/1(dout) -> pol1_in5_tap3/1(din)
  pol1_in5_tap2/2(sync_out) -> pol1_in5_tap3/2(sync)
  pol1_in5_tap2/3(coeff_out) -> pol1_in5_tap3/3(coeff)
  pol1_in5_tap2/4(taps_out) -> adder_1_5/3(din2)
  pol1_in5_tap3/1(dout) -> pol1_in5_tap4/1(din)
  pol1_in5_tap3/2(sync_out) -> pol1_in5_tap4/2(sync)
  pol1_in5_tap3/3(coeff_out) -> pol1_in5_tap4/3(coeff)
  pol1_in5_tap3/4(taps_out) -> adder_1_5/4(din3)
  pol1_in5_tap4/1(dout) -> pol1_in5_tap5/1(din)
  pol1_in5_tap4/2(sync_out) -> pol1_in5_tap5/2(sync)
  pol1_in5_tap4/3(coeff_out) -> pol1_in5_tap5/3(coeff)
  pol1_in5_tap4/4(taps_out) -> adder_1_5/5(din4)
  pol1_in5_tap5/1(dout) -> pol1_in5_tap6/1(din)
  pol1_in5_tap5/2(sync_out) -> pol1_in5_tap6/2(sync)
  pol1_in5_tap5/3(coeff_out) -> pol1_in5_tap6/3(coeff)
  pol1_in5_tap5/4(taps_out) -> adder_1_5/6(din5)
  pol1_in5_tap6/1(dout) -> pol1_in5_tap7/1(din)
  pol1_in5_tap6/2(sync_out) -> pol1_in5_tap7/2(sync)
  pol1_in5_tap6/3(coeff_out) -> pol1_in5_tap7/3(coeff)
  pol1_in5_tap6/4(taps_out) -> adder_1_5/7(din6)
  pol1_in5_last_tap/2(sync_out) -> adder_1_5/1(sync)
  pol1_in5_last_tap/1(tap_out) -> adder_1_5/9(din8)
  pol1_in5_tap7/1(dout) -> pol1_in5_last_tap/1(din)
  pol1_in5_tap7/2(sync_out) -> pol1_in5_last_tap/2(sync)
  pol1_in5_tap7/3(coeff_out) -> pol1_in5_last_tap/3(coeff)
  pol1_in5_tap7/4(taps_out) -> adder_1_5/8(din7)
  pol1_in6_first_tap/1(dout) -> pol1_in6_tap2/1(din)
  pol1_in6_first_tap/2(sync_out) -> pol1_in6_tap2/2(sync)
  pol1_in6_first_tap/3(coeff_out) -> pol1_in6_tap2/3(coeff)
  pol1_in6_first_tap/4(taps_out) -> adder_1_6/2(din1)
  pol1_in6_tap2/1(dout) -> pol1_in6_tap3/1(din)
  pol1_in6_tap2/2(sync_out) -> pol1_in6_tap3/2(sync)
  pol1_in6_tap2/3(coeff_out) -> pol1_in6_tap3/3(coeff)
  pol1_in6_tap2/4(taps_out) -> adder_1_6/3(din2)
  pol1_in6_tap3/1(dout) -> pol1_in6_tap4/1(din)
  pol1_in6_tap3/2(sync_out) -> pol1_in6_tap4/2(sync)
  pol1_in6_tap3/3(coeff_out) -> pol1_in6_tap4/3(coeff)
  pol1_in6_tap3/4(taps_out) -> adder_1_6/4(din3)
  pol1_in6_tap4/1(dout) -> pol1_in6_tap5/1(din)
  pol1_in6_tap4/2(sync_out) -> pol1_in6_tap5/2(sync)
  pol1_in6_tap4/3(coeff_out) -> pol1_in6_tap5/3(coeff)
  pol1_in6_tap4/4(taps_out) -> adder_1_6/5(din4)
  pol1_in6_tap5/1(dout) -> pol1_in6_tap6/1(din)
  pol1_in6_tap5/2(sync_out) -> pol1_in6_tap6/2(sync)
  pol1_in6_tap5/3(coeff_out) -> pol1_in6_tap6/3(coeff)
  pol1_in6_tap5/4(taps_out) -> adder_1_6/6(din5)
  pol1_in6_tap6/1(dout) -> pol1_in6_tap7/1(din)
  pol1_in6_tap6/2(sync_out) -> pol1_in6_tap7/2(sync)
  pol1_in6_tap6/3(coeff_out) -> pol1_in6_tap7/3(coeff)
  pol1_in6_tap6/4(taps_out) -> adder_1_6/7(din6)
  pol1_in6_last_tap/2(sync_out) -> adder_1_6/1(sync)
  pol1_in6_last_tap/1(tap_out) -> adder_1_6/9(din8)
  pol1_in6_tap7/1(dout) -> pol1_in6_last_tap/1(din)
  pol1_in6_tap7/2(sync_out) -> pol1_in6_last_tap/2(sync)
  pol1_in6_tap7/3(coeff_out) -> pol1_in6_last_tap/3(coeff)
  pol1_in6_tap7/4(taps_out) -> adder_1_6/8(din7)
  pol1_in7_first_tap/1(dout) -> pol1_in7_tap2/1(din)
  pol1_in7_first_tap/2(sync_out) -> pol1_in7_tap2/2(sync)
  pol1_in7_first_tap/3(coeff_out) -> pol1_in7_tap2/3(coeff)
  pol1_in7_first_tap/4(taps_out) -> adder_1_7/2(din1)
  pol1_in7_tap2/1(dout) -> pol1_in7_tap3/1(din)
  pol1_in7_tap2/2(sync_out) -> pol1_in7_tap3/2(sync)
  pol1_in7_tap2/3(coeff_out) -> pol1_in7_tap3/3(coeff)
  pol1_in7_tap2/4(taps_out) -> adder_1_7/3(din2)
  pol1_in7_tap3/1(dout) -> pol1_in7_tap4/1(din)
  pol1_in7_tap3/2(sync_out) -> pol1_in7_tap4/2(sync)
  pol1_in7_tap3/3(coeff_out) -> pol1_in7_tap4/3(coeff)
  pol1_in7_tap3/4(taps_out) -> adder_1_7/4(din3)
  pol1_in7_tap4/1(dout) -> pol1_in7_tap5/1(din)
  pol1_in7_tap4/2(sync_out) -> pol1_in7_tap5/2(sync)
  pol1_in7_tap4/3(coeff_out) -> pol1_in7_tap5/3(coeff)
  pol1_in7_tap4/4(taps_out) -> adder_1_7/5(din4)
  pol1_in7_tap5/1(dout) -> pol1_in7_tap6/1(din)
  pol1_in7_tap5/2(sync_out) -> pol1_in7_tap6/2(sync)
  pol1_in7_tap5/3(coeff_out) -> pol1_in7_tap6/3(coeff)
  pol1_in7_tap5/4(taps_out) -> adder_1_7/6(din5)
  pol1_in7_tap6/1(dout) -> pol1_in7_tap7/1(din)
  pol1_in7_tap6/2(sync_out) -> pol1_in7_tap7/2(sync)
  pol1_in7_tap6/3(coeff_out) -> pol1_in7_tap7/3(coeff)
  pol1_in7_tap6/4(taps_out) -> adder_1_7/7(din6)
  pol1_in7_last_tap/2(sync_out) -> adder_1_7/1(sync)
  pol1_in7_last_tap/1(tap_out) -> adder_1_7/9(din8)
  pol1_in7_tap7/1(dout) -> pol1_in7_last_tap/1(din)
  pol1_in7_tap7/2(sync_out) -> pol1_in7_last_tap/2(sync)
  pol1_in7_tap7/3(coeff_out) -> pol1_in7_last_tap/3(coeff)
  pol1_in7_tap7/4(taps_out) -> adder_1_7/8(din7)
  pol1_in8_first_tap/1(dout) -> pol1_in8_tap2/1(din)
  pol1_in8_first_tap/2(sync_out) -> pol1_in8_tap2/2(sync)
  pol1_in8_first_tap/3(coeff_out) -> pol1_in8_tap2/3(coeff)
  pol1_in8_first_tap/4(taps_out) -> adder_1_8/2(din1)
  pol1_in8_tap2/1(dout) -> pol1_in8_tap3/1(din)
  pol1_in8_tap2/2(sync_out) -> pol1_in8_tap3/2(sync)
  pol1_in8_tap2/3(coeff_out) -> pol1_in8_tap3/3(coeff)
  pol1_in8_tap2/4(taps_out) -> adder_1_8/3(din2)
  pol1_in8_tap3/1(dout) -> pol1_in8_tap4/1(din)
  pol1_in8_tap3/2(sync_out) -> pol1_in8_tap4/2(sync)
  pol1_in8_tap3/3(coeff_out) -> pol1_in8_tap4/3(coeff)
  pol1_in8_tap3/4(taps_out) -> adder_1_8/4(din3)
  pol1_in8_tap4/1(dout) -> pol1_in8_tap5/1(din)
  pol1_in8_tap4/2(sync_out) -> pol1_in8_tap5/2(sync)
  pol1_in8_tap4/3(coeff_out) -> pol1_in8_tap5/3(coeff)
  pol1_in8_tap4/4(taps_out) -> adder_1_8/5(din4)
  pol1_in8_tap5/1(dout) -> pol1_in8_tap6/1(din)
  pol1_in8_tap5/2(sync_out) -> pol1_in8_tap6/2(sync)
  pol1_in8_tap5/3(coeff_out) -> pol1_in8_tap6/3(coeff)
  pol1_in8_tap5/4(taps_out) -> adder_1_8/6(din5)
  pol1_in8_tap6/1(dout) -> pol1_in8_tap7/1(din)
  pol1_in8_tap6/2(sync_out) -> pol1_in8_tap7/2(sync)
  pol1_in8_tap6/3(coeff_out) -> pol1_in8_tap7/3(coeff)
  pol1_in8_tap6/4(taps_out) -> adder_1_8/7(din6)
  pol1_in8_last_tap/2(sync_out) -> adder_1_8/1(sync)
  pol1_in8_last_tap/1(tap_out) -> adder_1_8/9(din8)
  pol1_in8_tap7/1(dout) -> pol1_in8_last_tap/1(din)
  pol1_in8_tap7/2(sync_out) -> pol1_in8_last_tap/2(sync)
  pol1_in8_tap7/3(coeff_out) -> pol1_in8_last_tap/3(coeff)
  pol1_in8_tap7/4(taps_out) -> adder_1_8/8(din7)
  pol1_in9_first_tap/1(dout) -> pol1_in9_tap2/1(din)
  pol1_in9_first_tap/2(sync_out) -> pol1_in9_tap2/2(sync)
  pol1_in9_first_tap/3(coeff_out) -> pol1_in9_tap2/3(coeff)
  pol1_in9_first_tap/4(taps_out) -> adder_1_9/2(din1)
  pol1_in9_tap2/1(dout) -> pol1_in9_tap3/1(din)
  pol1_in9_tap2/2(sync_out) -> pol1_in9_tap3/2(sync)
  pol1_in9_tap2/3(coeff_out) -> pol1_in9_tap3/3(coeff)
  pol1_in9_tap2/4(taps_out) -> adder_1_9/3(din2)
  pol1_in9_tap3/1(dout) -> pol1_in9_tap4/1(din)
  pol1_in9_tap3/2(sync_out) -> pol1_in9_tap4/2(sync)
  pol1_in9_tap3/3(coeff_out) -> pol1_in9_tap4/3(coeff)
  pol1_in9_tap3/4(taps_out) -> adder_1_9/4(din3)
  pol1_in9_tap4/1(dout) -> pol1_in9_tap5/1(din)
  pol1_in9_tap4/2(sync_out) -> pol1_in9_tap5/2(sync)
  pol1_in9_tap4/3(coeff_out) -> pol1_in9_tap5/3(coeff)
  pol1_in9_tap4/4(taps_out) -> adder_1_9/5(din4)
  pol1_in9_tap5/1(dout) -> pol1_in9_tap6/1(din)
  pol1_in9_tap5/2(sync_out) -> pol1_in9_tap6/2(sync)
  pol1_in9_tap5/3(coeff_out) -> pol1_in9_tap6/3(coeff)
  pol1_in9_tap5/4(taps_out) -> adder_1_9/6(din5)
  pol1_in9_tap6/1(dout) -> pol1_in9_tap7/1(din)
  pol1_in9_tap6/2(sync_out) -> pol1_in9_tap7/2(sync)
  pol1_in9_tap6/3(coeff_out) -> pol1_in9_tap7/3(coeff)
  pol1_in9_tap6/4(taps_out) -> adder_1_9/7(din6)
  pol1_in9_last_tap/2(sync_out) -> adder_1_9/1(sync)
  pol1_in9_last_tap/1(tap_out) -> adder_1_9/9(din8)
  pol1_in9_tap7/1(dout) -> pol1_in9_last_tap/1(din)
  pol1_in9_tap7/2(sync_out) -> pol1_in9_last_tap/2(sync)
  pol1_in9_tap7/3(coeff_out) -> pol1_in9_last_tap/3(coeff)
  pol1_in9_tap7/4(taps_out) -> adder_1_9/8(din7)
  pol1_in10_first_tap/1(dout) -> pol1_in10_tap2/1(din)
  pol1_in10_first_tap/2(sync_out) -> pol1_in10_tap2/2(sync)
  pol1_in10_first_tap/3(coeff_out) -> pol1_in10_tap2/3(coeff)
  pol1_in10_first_tap/4(taps_out) -> adder_1_10/2(din1)
  pol1_in10_tap2/1(dout) -> pol1_in10_tap3/1(din)
  pol1_in10_tap2/2(sync_out) -> pol1_in10_tap3/2(sync)
  pol1_in10_tap2/3(coeff_out) -> pol1_in10_tap3/3(coeff)
  pol1_in10_tap2/4(taps_out) -> adder_1_10/3(din2)
  pol1_in10_tap3/1(dout) -> pol1_in10_tap4/1(din)
  pol1_in10_tap3/2(sync_out) -> pol1_in10_tap4/2(sync)
  pol1_in10_tap3/3(coeff_out) -> pol1_in10_tap4/3(coeff)
  pol1_in10_tap3/4(taps_out) -> adder_1_10/4(din3)
  pol1_in10_tap4/1(dout) -> pol1_in10_tap5/1(din)
  pol1_in10_tap4/2(sync_out) -> pol1_in10_tap5/2(sync)
  pol1_in10_tap4/3(coeff_out) -> pol1_in10_tap5/3(coeff)
  pol1_in10_tap4/4(taps_out) -> adder_1_10/5(din4)
  pol1_in10_tap5/1(dout) -> pol1_in10_tap6/1(din)
  pol1_in10_tap5/2(sync_out) -> pol1_in10_tap6/2(sync)
  pol1_in10_tap5/3(coeff_out) -> pol1_in10_tap6/3(coeff)
  pol1_in10_tap5/4(taps_out) -> adder_1_10/6(din5)
  pol1_in10_tap6/1(dout) -> pol1_in10_tap7/1(din)
  pol1_in10_tap6/2(sync_out) -> pol1_in10_tap7/2(sync)
  pol1_in10_tap6/3(coeff_out) -> pol1_in10_tap7/3(coeff)
  pol1_in10_tap6/4(taps_out) -> adder_1_10/7(din6)
  pol1_in10_last_tap/2(sync_out) -> adder_1_10/1(sync)
  pol1_in10_last_tap/1(tap_out) -> adder_1_10/9(din8)
  pol1_in10_tap7/1(dout) -> pol1_in10_last_tap/1(din)
  pol1_in10_tap7/2(sync_out) -> pol1_in10_last_tap/2(sync)
  pol1_in10_tap7/3(coeff_out) -> pol1_in10_last_tap/3(coeff)
  pol1_in10_tap7/4(taps_out) -> adder_1_10/8(din7)
  pol1_in11_first_tap/1(dout) -> pol1_in11_tap2/1(din)
  pol1_in11_first_tap/2(sync_out) -> pol1_in11_tap2/2(sync)
  pol1_in11_first_tap/3(coeff_out) -> pol1_in11_tap2/3(coeff)
  pol1_in11_first_tap/4(taps_out) -> adder_1_11/2(din1)
  pol1_in11_tap2/1(dout) -> pol1_in11_tap3/1(din)
  pol1_in11_tap2/2(sync_out) -> pol1_in11_tap3/2(sync)
  pol1_in11_tap2/3(coeff_out) -> pol1_in11_tap3/3(coeff)
  pol1_in11_tap2/4(taps_out) -> adder_1_11/3(din2)
  pol1_in11_tap3/1(dout) -> pol1_in11_tap4/1(din)
  pol1_in11_tap3/2(sync_out) -> pol1_in11_tap4/2(sync)
  pol1_in11_tap3/3(coeff_out) -> pol1_in11_tap4/3(coeff)
  pol1_in11_tap3/4(taps_out) -> adder_1_11/4(din3)
  pol1_in11_tap4/1(dout) -> pol1_in11_tap5/1(din)
  pol1_in11_tap4/2(sync_out) -> pol1_in11_tap5/2(sync)
  pol1_in11_tap4/3(coeff_out) -> pol1_in11_tap5/3(coeff)
  pol1_in11_tap4/4(taps_out) -> adder_1_11/5(din4)
  pol1_in11_tap5/1(dout) -> pol1_in11_tap6/1(din)
  pol1_in11_tap5/2(sync_out) -> pol1_in11_tap6/2(sync)
  pol1_in11_tap5/3(coeff_out) -> pol1_in11_tap6/3(coeff)
  pol1_in11_tap5/4(taps_out) -> adder_1_11/6(din5)
  pol1_in11_tap6/1(dout) -> pol1_in11_tap7/1(din)
  pol1_in11_tap6/2(sync_out) -> pol1_in11_tap7/2(sync)
  pol1_in11_tap6/3(coeff_out) -> pol1_in11_tap7/3(coeff)
  pol1_in11_tap6/4(taps_out) -> adder_1_11/7(din6)
  pol1_in11_last_tap/2(sync_out) -> adder_1_11/1(sync)
  pol1_in11_last_tap/1(tap_out) -> adder_1_11/9(din8)
  pol1_in11_tap7/1(dout) -> pol1_in11_last_tap/1(din)
  pol1_in11_tap7/2(sync_out) -> pol1_in11_last_tap/2(sync)
  pol1_in11_tap7/3(coeff_out) -> pol1_in11_last_tap/3(coeff)
  pol1_in11_tap7/4(taps_out) -> adder_1_11/8(din7)
  pol1_in12_first_tap/1(dout) -> pol1_in12_tap2/1(din)
  pol1_in12_first_tap/2(sync_out) -> pol1_in12_tap2/2(sync)
  pol1_in12_first_tap/3(coeff_out) -> pol1_in12_tap2/3(coeff)
  pol1_in12_first_tap/4(taps_out) -> adder_1_12/2(din1)
  pol1_in12_tap2/1(dout) -> pol1_in12_tap3/1(din)
  pol1_in12_tap2/2(sync_out) -> pol1_in12_tap3/2(sync)
  pol1_in12_tap2/3(coeff_out) -> pol1_in12_tap3/3(coeff)
  pol1_in12_tap2/4(taps_out) -> adder_1_12/3(din2)
  pol1_in12_tap3/1(dout) -> pol1_in12_tap4/1(din)
  pol1_in12_tap3/2(sync_out) -> pol1_in12_tap4/2(sync)
  pol1_in12_tap3/3(coeff_out) -> pol1_in12_tap4/3(coeff)
  pol1_in12_tap3/4(taps_out) -> adder_1_12/4(din3)
  pol1_in12_tap4/1(dout) -> pol1_in12_tap5/1(din)
  pol1_in12_tap4/2(sync_out) -> pol1_in12_tap5/2(sync)
  pol1_in12_tap4/3(coeff_out) -> pol1_in12_tap5/3(coeff)
  pol1_in12_tap4/4(taps_out) -> adder_1_12/5(din4)
  pol1_in12_tap5/1(dout) -> pol1_in12_tap6/1(din)
  pol1_in12_tap5/2(sync_out) -> pol1_in12_tap6/2(sync)
  pol1_in12_tap5/3(coeff_out) -> pol1_in12_tap6/3(coeff)
  pol1_in12_tap5/4(taps_out) -> adder_1_12/6(din5)
  pol1_in12_tap6/1(dout) -> pol1_in12_tap7/1(din)
  pol1_in12_tap6/2(sync_out) -> pol1_in12_tap7/2(sync)
  pol1_in12_tap6/3(coeff_out) -> pol1_in12_tap7/3(coeff)
  pol1_in12_tap6/4(taps_out) -> adder_1_12/7(din6)
  pol1_in12_last_tap/2(sync_out) -> adder_1_12/1(sync)
  pol1_in12_last_tap/1(tap_out) -> adder_1_12/9(din8)
  pol1_in12_tap7/1(dout) -> pol1_in12_last_tap/1(din)
  pol1_in12_tap7/2(sync_out) -> pol1_in12_last_tap/2(sync)
  pol1_in12_tap7/3(coeff_out) -> pol1_in12_last_tap/3(coeff)
  pol1_in12_tap7/4(taps_out) -> adder_1_12/8(din7)
  pol1_in13_first_tap/1(dout) -> pol1_in13_tap2/1(din)
  pol1_in13_first_tap/2(sync_out) -> pol1_in13_tap2/2(sync)
  pol1_in13_first_tap/3(coeff_out) -> pol1_in13_tap2/3(coeff)
  pol1_in13_first_tap/4(taps_out) -> adder_1_13/2(din1)
  pol1_in13_tap2/1(dout) -> pol1_in13_tap3/1(din)
  pol1_in13_tap2/2(sync_out) -> pol1_in13_tap3/2(sync)
  pol1_in13_tap2/3(coeff_out) -> pol1_in13_tap3/3(coeff)
  pol1_in13_tap2/4(taps_out) -> adder_1_13/3(din2)
  pol1_in13_tap3/1(dout) -> pol1_in13_tap4/1(din)
  pol1_in13_tap3/2(sync_out) -> pol1_in13_tap4/2(sync)
  pol1_in13_tap3/3(coeff_out) -> pol1_in13_tap4/3(coeff)
  pol1_in13_tap3/4(taps_out) -> adder_1_13/4(din3)
  pol1_in13_tap4/1(dout) -> pol1_in13_tap5/1(din)
  pol1_in13_tap4/2(sync_out) -> pol1_in13_tap5/2(sync)
  pol1_in13_tap4/3(coeff_out) -> pol1_in13_tap5/3(coeff)
  pol1_in13_tap4/4(taps_out) -> adder_1_13/5(din4)
  pol1_in13_tap5/1(dout) -> pol1_in13_tap6/1(din)
  pol1_in13_tap5/2(sync_out) -> pol1_in13_tap6/2(sync)
  pol1_in13_tap5/3(coeff_out) -> pol1_in13_tap6/3(coeff)
  pol1_in13_tap5/4(taps_out) -> adder_1_13/6(din5)
  pol1_in13_tap6/1(dout) -> pol1_in13_tap7/1(din)
  pol1_in13_tap6/2(sync_out) -> pol1_in13_tap7/2(sync)
  pol1_in13_tap6/3(coeff_out) -> pol1_in13_tap7/3(coeff)
  pol1_in13_tap6/4(taps_out) -> adder_1_13/7(din6)
  pol1_in13_last_tap/2(sync_out) -> adder_1_13/1(sync)
  pol1_in13_last_tap/1(tap_out) -> adder_1_13/9(din8)
  pol1_in13_tap7/1(dout) -> pol1_in13_last_tap/1(din)
  pol1_in13_tap7/2(sync_out) -> pol1_in13_last_tap/2(sync)
  pol1_in13_tap7/3(coeff_out) -> pol1_in13_last_tap/3(coeff)
  pol1_in13_tap7/4(taps_out) -> adder_1_13/8(din7)
  pol1_in14_first_tap/1(dout) -> pol1_in14_tap2/1(din)
  pol1_in14_first_tap/2(sync_out) -> pol1_in14_tap2/2(sync)
  pol1_in14_first_tap/3(coeff_out) -> pol1_in14_tap2/3(coeff)
  pol1_in14_first_tap/4(taps_out) -> adder_1_14/2(din1)
  pol1_in14_tap2/1(dout) -> pol1_in14_tap3/1(din)
  pol1_in14_tap2/2(sync_out) -> pol1_in14_tap3/2(sync)
  pol1_in14_tap2/3(coeff_out) -> pol1_in14_tap3/3(coeff)
  pol1_in14_tap2/4(taps_out) -> adder_1_14/3(din2)
  pol1_in14_tap3/1(dout) -> pol1_in14_tap4/1(din)
  pol1_in14_tap3/2(sync_out) -> pol1_in14_tap4/2(sync)
  pol1_in14_tap3/3(coeff_out) -> pol1_in14_tap4/3(coeff)
  pol1_in14_tap3/4(taps_out) -> adder_1_14/4(din3)
  pol1_in14_tap4/1(dout) -> pol1_in14_tap5/1(din)
  pol1_in14_tap4/2(sync_out) -> pol1_in14_tap5/2(sync)
  pol1_in14_tap4/3(coeff_out) -> pol1_in14_tap5/3(coeff)
  pol1_in14_tap4/4(taps_out) -> adder_1_14/5(din4)
  pol1_in14_tap5/1(dout) -> pol1_in14_tap6/1(din)
  pol1_in14_tap5/2(sync_out) -> pol1_in14_tap6/2(sync)
  pol1_in14_tap5/3(coeff_out) -> pol1_in14_tap6/3(coeff)
  pol1_in14_tap5/4(taps_out) -> adder_1_14/6(din5)
  pol1_in14_tap6/1(dout) -> pol1_in14_tap7/1(din)
  pol1_in14_tap6/2(sync_out) -> pol1_in14_tap7/2(sync)
  pol1_in14_tap6/3(coeff_out) -> pol1_in14_tap7/3(coeff)
  pol1_in14_tap6/4(taps_out) -> adder_1_14/7(din6)
  pol1_in14_last_tap/2(sync_out) -> adder_1_14/1(sync)
  pol1_in14_last_tap/1(tap_out) -> adder_1_14/9(din8)
  pol1_in14_tap7/1(dout) -> pol1_in14_last_tap/1(din)
  pol1_in14_tap7/2(sync_out) -> pol1_in14_last_tap/2(sync)
  pol1_in14_tap7/3(coeff_out) -> pol1_in14_last_tap/3(coeff)
  pol1_in14_tap7/4(taps_out) -> adder_1_14/8(din7)
  pol1_in15_first_tap/1(dout) -> pol1_in15_tap2/1(din)
  pol1_in15_first_tap/2(sync_out) -> pol1_in15_tap2/2(sync)
  pol1_in15_first_tap/3(coeff_out) -> pol1_in15_tap2/3(coeff)
  pol1_in15_first_tap/4(taps_out) -> adder_1_15/2(din1)
  pol1_in15_tap2/1(dout) -> pol1_in15_tap3/1(din)
  pol1_in15_tap2/2(sync_out) -> pol1_in15_tap3/2(sync)
  pol1_in15_tap2/3(coeff_out) -> pol1_in15_tap3/3(coeff)
  pol1_in15_tap2/4(taps_out) -> adder_1_15/3(din2)
  pol1_in15_tap3/1(dout) -> pol1_in15_tap4/1(din)
  pol1_in15_tap3/2(sync_out) -> pol1_in15_tap4/2(sync)
  pol1_in15_tap3/3(coeff_out) -> pol1_in15_tap4/3(coeff)
  pol1_in15_tap3/4(taps_out) -> adder_1_15/4(din3)
  pol1_in15_tap4/1(dout) -> pol1_in15_tap5/1(din)
  pol1_in15_tap4/2(sync_out) -> pol1_in15_tap5/2(sync)
  pol1_in15_tap4/3(coeff_out) -> pol1_in15_tap5/3(coeff)
  pol1_in15_tap4/4(taps_out) -> adder_1_15/5(din4)
  pol1_in15_tap5/1(dout) -> pol1_in15_tap6/1(din)
  pol1_in15_tap5/2(sync_out) -> pol1_in15_tap6/2(sync)
  pol1_in15_tap5/3(coeff_out) -> pol1_in15_tap6/3(coeff)
  pol1_in15_tap5/4(taps_out) -> adder_1_15/6(din5)
  pol1_in15_tap6/1(dout) -> pol1_in15_tap7/1(din)
  pol1_in15_tap6/2(sync_out) -> pol1_in15_tap7/2(sync)
  pol1_in15_tap6/3(coeff_out) -> pol1_in15_tap7/3(coeff)
  pol1_in15_tap6/4(taps_out) -> adder_1_15/7(din6)
  pol1_in15_last_tap/2(sync_out) -> adder_1_15/1(sync)
  pol1_in15_last_tap/1(tap_out) -> adder_1_15/9(din8)
  pol1_in15_tap7/1(dout) -> pol1_in15_last_tap/1(din)
  pol1_in15_tap7/2(sync_out) -> pol1_in15_last_tap/2(sync)
  pol1_in15_tap7/3(coeff_out) -> pol1_in15_last_tap/3(coeff)
  pol1_in15_tap7/4(taps_out) -> adder_1_15/8(din7)
  pol1_in16_first_tap/1(dout) -> pol1_in16_tap2/1(din)
  pol1_in16_first_tap/2(sync_out) -> pol1_in16_tap2/2(sync)
  pol1_in16_first_tap/3(coeff_out) -> pol1_in16_tap2/3(coeff)
  pol1_in16_first_tap/4(taps_out) -> adder_1_16/2(din1)
  pol1_in16_tap2/1(dout) -> pol1_in16_tap3/1(din)
  pol1_in16_tap2/2(sync_out) -> pol1_in16_tap3/2(sync)
  pol1_in16_tap2/3(coeff_out) -> pol1_in16_tap3/3(coeff)
  pol1_in16_tap2/4(taps_out) -> adder_1_16/3(din2)
  pol1_in16_tap3/1(dout) -> pol1_in16_tap4/1(din)
  pol1_in16_tap3/2(sync_out) -> pol1_in16_tap4/2(sync)
  pol1_in16_tap3/3(coeff_out) -> pol1_in16_tap4/3(coeff)
  pol1_in16_tap3/4(taps_out) -> adder_1_16/4(din3)
  pol1_in16_tap4/1(dout) -> pol1_in16_tap5/1(din)
  pol1_in16_tap4/2(sync_out) -> pol1_in16_tap5/2(sync)
  pol1_in16_tap4/3(coeff_out) -> pol1_in16_tap5/3(coeff)
  pol1_in16_tap4/4(taps_out) -> adder_1_16/5(din4)
  pol1_in16_tap5/1(dout) -> pol1_in16_tap6/1(din)
  pol1_in16_tap5/2(sync_out) -> pol1_in16_tap6/2(sync)
  pol1_in16_tap5/3(coeff_out) -> pol1_in16_tap6/3(coeff)
  pol1_in16_tap5/4(taps_out) -> adder_1_16/6(din5)
  pol1_in16_tap6/1(dout) -> pol1_in16_tap7/1(din)
  pol1_in16_tap6/2(sync_out) -> pol1_in16_tap7/2(sync)
  pol1_in16_tap6/3(coeff_out) -> pol1_in16_tap7/3(coeff)
  pol1_in16_tap6/4(taps_out) -> adder_1_16/7(din6)
  pol1_in16_last_tap/2(sync_out) -> adder_1_16/1(sync)
  pol1_in16_last_tap/1(tap_out) -> adder_1_16/9(din8)
  pol1_in16_tap7/1(dout) -> pol1_in16_last_tap/1(din)
  pol1_in16_tap7/2(sync_out) -> pol1_in16_last_tap/2(sync)
  pol1_in16_tap7/3(coeff_out) -> pol1_in16_last_tap/3(coeff)
  pol1_in16_tap7/4(taps_out) -> adder_1_16/8(din7)
  pol1_in17_first_tap/1(dout) -> pol1_in17_tap2/1(din)
  pol1_in17_first_tap/2(sync_out) -> pol1_in17_tap2/2(sync)
  pol1_in17_first_tap/3(coeff_out) -> pol1_in17_tap2/3(coeff)
  pol1_in17_first_tap/4(taps_out) -> adder_1_17/2(din1)
  pol1_in17_tap2/1(dout) -> pol1_in17_tap3/1(din)
  pol1_in17_tap2/2(sync_out) -> pol1_in17_tap3/2(sync)
  pol1_in17_tap2/3(coeff_out) -> pol1_in17_tap3/3(coeff)
  pol1_in17_tap2/4(taps_out) -> adder_1_17/3(din2)
  pol1_in17_tap3/1(dout) -> pol1_in17_tap4/1(din)
  pol1_in17_tap3/2(sync_out) -> pol1_in17_tap4/2(sync)
  pol1_in17_tap3/3(coeff_out) -> pol1_in17_tap4/3(coeff)
  pol1_in17_tap3/4(taps_out) -> adder_1_17/4(din3)
  pol1_in17_tap4/1(dout) -> pol1_in17_tap5/1(din)
  pol1_in17_tap4/2(sync_out) -> pol1_in17_tap5/2(sync)
  pol1_in17_tap4/3(coeff_out) -> pol1_in17_tap5/3(coeff)
  pol1_in17_tap4/4(taps_out) -> adder_1_17/5(din4)
  pol1_in17_tap5/1(dout) -> pol1_in17_tap6/1(din)
  pol1_in17_tap5/2(sync_out) -> pol1_in17_tap6/2(sync)
  pol1_in17_tap5/3(coeff_out) -> pol1_in17_tap6/3(coeff)
  pol1_in17_tap5/4(taps_out) -> adder_1_17/6(din5)
  pol1_in17_tap6/1(dout) -> pol1_in17_tap7/1(din)
  pol1_in17_tap6/2(sync_out) -> pol1_in17_tap7/2(sync)
  pol1_in17_tap6/3(coeff_out) -> pol1_in17_tap7/3(coeff)
  pol1_in17_tap6/4(taps_out) -> adder_1_17/7(din6)
  pol1_in17_last_tap/2(sync_out) -> adder_1_17/1(sync)
  pol1_in17_last_tap/1(tap_out) -> adder_1_17/9(din8)
  pol1_in17_tap7/1(dout) -> pol1_in17_last_tap/1(din)
  pol1_in17_tap7/2(sync_out) -> pol1_in17_last_tap/2(sync)
  pol1_in17_tap7/3(coeff_out) -> pol1_in17_last_tap/3(coeff)
  pol1_in17_tap7/4(taps_out) -> adder_1_17/8(din7)
  pol1_in18_first_tap/1(dout) -> pol1_in18_tap2/1(din)
  pol1_in18_first_tap/2(sync_out) -> pol1_in18_tap2/2(sync)
  pol1_in18_first_tap/3(coeff_out) -> pol1_in18_tap2/3(coeff)
  pol1_in18_first_tap/4(taps_out) -> adder_1_18/2(din1)
  pol1_in18_tap2/1(dout) -> pol1_in18_tap3/1(din)
  pol1_in18_tap2/2(sync_out) -> pol1_in18_tap3/2(sync)
  pol1_in18_tap2/3(coeff_out) -> pol1_in18_tap3/3(coeff)
  pol1_in18_tap2/4(taps_out) -> adder_1_18/3(din2)
  pol1_in18_tap3/1(dout) -> pol1_in18_tap4/1(din)
  pol1_in18_tap3/2(sync_out) -> pol1_in18_tap4/2(sync)
  pol1_in18_tap3/3(coeff_out) -> pol1_in18_tap4/3(coeff)
  pol1_in18_tap3/4(taps_out) -> adder_1_18/4(din3)
  pol1_in18_tap4/1(dout) -> pol1_in18_tap5/1(din)
  pol1_in18_tap4/2(sync_out) -> pol1_in18_tap5/2(sync)
  pol1_in18_tap4/3(coeff_out) -> pol1_in18_tap5/3(coeff)
  pol1_in18_tap4/4(taps_out) -> adder_1_18/5(din4)
  pol1_in18_tap5/1(dout) -> pol1_in18_tap6/1(din)
  pol1_in18_tap5/2(sync_out) -> pol1_in18_tap6/2(sync)
  pol1_in18_tap5/3(coeff_out) -> pol1_in18_tap6/3(coeff)
  pol1_in18_tap5/4(taps_out) -> adder_1_18/6(din5)
  pol1_in18_tap6/1(dout) -> pol1_in18_tap7/1(din)
  pol1_in18_tap6/2(sync_out) -> pol1_in18_tap7/2(sync)
  pol1_in18_tap6/3(coeff_out) -> pol1_in18_tap7/3(coeff)
  pol1_in18_tap6/4(taps_out) -> adder_1_18/7(din6)
  pol1_in18_last_tap/2(sync_out) -> adder_1_18/1(sync)
  pol1_in18_last_tap/1(tap_out) -> adder_1_18/9(din8)
  pol1_in18_tap7/1(dout) -> pol1_in18_last_tap/1(din)
  pol1_in18_tap7/2(sync_out) -> pol1_in18_last_tap/2(sync)
  pol1_in18_tap7/3(coeff_out) -> pol1_in18_last_tap/3(coeff)
  pol1_in18_tap7/4(taps_out) -> adder_1_18/8(din7)
  pol1_in19_first_tap/1(dout) -> pol1_in19_tap2/1(din)
  pol1_in19_first_tap/2(sync_out) -> pol1_in19_tap2/2(sync)
  pol1_in19_first_tap/3(coeff_out) -> pol1_in19_tap2/3(coeff)
  pol1_in19_first_tap/4(taps_out) -> adder_1_19/2(din1)
  pol1_in19_tap2/1(dout) -> pol1_in19_tap3/1(din)
  pol1_in19_tap2/2(sync_out) -> pol1_in19_tap3/2(sync)
  pol1_in19_tap2/3(coeff_out) -> pol1_in19_tap3/3(coeff)
  pol1_in19_tap2/4(taps_out) -> adder_1_19/3(din2)
  pol1_in19_tap3/1(dout) -> pol1_in19_tap4/1(din)
  pol1_in19_tap3/2(sync_out) -> pol1_in19_tap4/2(sync)
  pol1_in19_tap3/3(coeff_out) -> pol1_in19_tap4/3(coeff)
  pol1_in19_tap3/4(taps_out) -> adder_1_19/4(din3)
  pol1_in19_tap4/1(dout) -> pol1_in19_tap5/1(din)
  pol1_in19_tap4/2(sync_out) -> pol1_in19_tap5/2(sync)
  pol1_in19_tap4/3(coeff_out) -> pol1_in19_tap5/3(coeff)
  pol1_in19_tap4/4(taps_out) -> adder_1_19/5(din4)
  pol1_in19_tap5/1(dout) -> pol1_in19_tap6/1(din)
  pol1_in19_tap5/2(sync_out) -> pol1_in19_tap6/2(sync)
  pol1_in19_tap5/3(coeff_out) -> pol1_in19_tap6/3(coeff)
  pol1_in19_tap5/4(taps_out) -> adder_1_19/6(din5)
  pol1_in19_tap6/1(dout) -> pol1_in19_tap7/1(din)
  pol1_in19_tap6/2(sync_out) -> pol1_in19_tap7/2(sync)
  pol1_in19_tap6/3(coeff_out) -> pol1_in19_tap7/3(coeff)
  pol1_in19_tap6/4(taps_out) -> adder_1_19/7(din6)
  pol1_in19_last_tap/2(sync_out) -> adder_1_19/1(sync)
  pol1_in19_last_tap/1(tap_out) -> adder_1_19/9(din8)
  pol1_in19_tap7/1(dout) -> pol1_in19_last_tap/1(din)
  pol1_in19_tap7/2(sync_out) -> pol1_in19_last_tap/2(sync)
  pol1_in19_tap7/3(coeff_out) -> pol1_in19_last_tap/3(coeff)
  pol1_in19_tap7/4(taps_out) -> adder_1_19/8(din7)
  pol1_in20_first_tap/1(dout) -> pol1_in20_tap2/1(din)
  pol1_in20_first_tap/2(sync_out) -> pol1_in20_tap2/2(sync)
  pol1_in20_first_tap/3(coeff_out) -> pol1_in20_tap2/3(coeff)
  pol1_in20_first_tap/4(taps_out) -> adder_1_20/2(din1)
  pol1_in20_tap2/1(dout) -> pol1_in20_tap3/1(din)
  pol1_in20_tap2/2(sync_out) -> pol1_in20_tap3/2(sync)
  pol1_in20_tap2/3(coeff_out) -> pol1_in20_tap3/3(coeff)
  pol1_in20_tap2/4(taps_out) -> adder_1_20/3(din2)
  pol1_in20_tap3/1(dout) -> pol1_in20_tap4/1(din)
  pol1_in20_tap3/2(sync_out) -> pol1_in20_tap4/2(sync)
  pol1_in20_tap3/3(coeff_out) -> pol1_in20_tap4/3(coeff)
  pol1_in20_tap3/4(taps_out) -> adder_1_20/4(din3)
  pol1_in20_tap4/1(dout) -> pol1_in20_tap5/1(din)
  pol1_in20_tap4/2(sync_out) -> pol1_in20_tap5/2(sync)
  pol1_in20_tap4/3(coeff_out) -> pol1_in20_tap5/3(coeff)
  pol1_in20_tap4/4(taps_out) -> adder_1_20/5(din4)
  pol1_in20_tap5/1(dout) -> pol1_in20_tap6/1(din)
  pol1_in20_tap5/2(sync_out) -> pol1_in20_tap6/2(sync)
  pol1_in20_tap5/3(coeff_out) -> pol1_in20_tap6/3(coeff)
  pol1_in20_tap5/4(taps_out) -> adder_1_20/6(din5)
  pol1_in20_tap6/1(dout) -> pol1_in20_tap7/1(din)
  pol1_in20_tap6/2(sync_out) -> pol1_in20_tap7/2(sync)
  pol1_in20_tap6/3(coeff_out) -> pol1_in20_tap7/3(coeff)
  pol1_in20_tap6/4(taps_out) -> adder_1_20/7(din6)
  pol1_in20_last_tap/2(sync_out) -> adder_1_20/1(sync)
  pol1_in20_last_tap/1(tap_out) -> adder_1_20/9(din8)
  pol1_in20_tap7/1(dout) -> pol1_in20_last_tap/1(din)
  pol1_in20_tap7/2(sync_out) -> pol1_in20_last_tap/2(sync)
  pol1_in20_tap7/3(coeff_out) -> pol1_in20_last_tap/3(coeff)
  pol1_in20_tap7/4(taps_out) -> adder_1_20/8(din7)
  pol1_in21_first_tap/1(dout) -> pol1_in21_tap2/1(din)
  pol1_in21_first_tap/2(sync_out) -> pol1_in21_tap2/2(sync)
  pol1_in21_first_tap/3(coeff_out) -> pol1_in21_tap2/3(coeff)
  pol1_in21_first_tap/4(taps_out) -> adder_1_21/2(din1)
  pol1_in21_tap2/1(dout) -> pol1_in21_tap3/1(din)
  pol1_in21_tap2/2(sync_out) -> pol1_in21_tap3/2(sync)
  pol1_in21_tap2/3(coeff_out) -> pol1_in21_tap3/3(coeff)
  pol1_in21_tap2/4(taps_out) -> adder_1_21/3(din2)
  pol1_in21_tap3/1(dout) -> pol1_in21_tap4/1(din)
  pol1_in21_tap3/2(sync_out) -> pol1_in21_tap4/2(sync)
  pol1_in21_tap3/3(coeff_out) -> pol1_in21_tap4/3(coeff)
  pol1_in21_tap3/4(taps_out) -> adder_1_21/4(din3)
  pol1_in21_tap4/1(dout) -> pol1_in21_tap5/1(din)
  pol1_in21_tap4/2(sync_out) -> pol1_in21_tap5/2(sync)
  pol1_in21_tap4/3(coeff_out) -> pol1_in21_tap5/3(coeff)
  pol1_in21_tap4/4(taps_out) -> adder_1_21/5(din4)
  pol1_in21_tap5/1(dout) -> pol1_in21_tap6/1(din)
  pol1_in21_tap5/2(sync_out) -> pol1_in21_tap6/2(sync)
  pol1_in21_tap5/3(coeff_out) -> pol1_in21_tap6/3(coeff)
  pol1_in21_tap5/4(taps_out) -> adder_1_21/6(din5)
  pol1_in21_tap6/1(dout) -> pol1_in21_tap7/1(din)
  pol1_in21_tap6/2(sync_out) -> pol1_in21_tap7/2(sync)
  pol1_in21_tap6/3(coeff_out) -> pol1_in21_tap7/3(coeff)
  pol1_in21_tap6/4(taps_out) -> adder_1_21/7(din6)
  pol1_in21_last_tap/2(sync_out) -> adder_1_21/1(sync)
  pol1_in21_last_tap/1(tap_out) -> adder_1_21/9(din8)
  pol1_in21_tap7/1(dout) -> pol1_in21_last_tap/1(din)
  pol1_in21_tap7/2(sync_out) -> pol1_in21_last_tap/2(sync)
  pol1_in21_tap7/3(coeff_out) -> pol1_in21_last_tap/3(coeff)
  pol1_in21_tap7/4(taps_out) -> adder_1_21/8(din7)
  pol1_in22_first_tap/1(dout) -> pol1_in22_tap2/1(din)
  pol1_in22_first_tap/2(sync_out) -> pol1_in22_tap2/2(sync)
  pol1_in22_first_tap/3(coeff_out) -> pol1_in22_tap2/3(coeff)
  pol1_in22_first_tap/4(taps_out) -> adder_1_22/2(din1)
  pol1_in22_tap2/1(dout) -> pol1_in22_tap3/1(din)
  pol1_in22_tap2/2(sync_out) -> pol1_in22_tap3/2(sync)
  pol1_in22_tap2/3(coeff_out) -> pol1_in22_tap3/3(coeff)
  pol1_in22_tap2/4(taps_out) -> adder_1_22/3(din2)
  pol1_in22_tap3/1(dout) -> pol1_in22_tap4/1(din)
  pol1_in22_tap3/2(sync_out) -> pol1_in22_tap4/2(sync)
  pol1_in22_tap3/3(coeff_out) -> pol1_in22_tap4/3(coeff)
  pol1_in22_tap3/4(taps_out) -> adder_1_22/4(din3)
  pol1_in22_tap4/1(dout) -> pol1_in22_tap5/1(din)
  pol1_in22_tap4/2(sync_out) -> pol1_in22_tap5/2(sync)
  pol1_in22_tap4/3(coeff_out) -> pol1_in22_tap5/3(coeff)
  pol1_in22_tap4/4(taps_out) -> adder_1_22/5(din4)
  pol1_in22_tap5/1(dout) -> pol1_in22_tap6/1(din)
  pol1_in22_tap5/2(sync_out) -> pol1_in22_tap6/2(sync)
  pol1_in22_tap5/3(coeff_out) -> pol1_in22_tap6/3(coeff)
  pol1_in22_tap5/4(taps_out) -> adder_1_22/6(din5)
  pol1_in22_tap6/1(dout) -> pol1_in22_tap7/1(din)
  pol1_in22_tap6/2(sync_out) -> pol1_in22_tap7/2(sync)
  pol1_in22_tap6/3(coeff_out) -> pol1_in22_tap7/3(coeff)
  pol1_in22_tap6/4(taps_out) -> adder_1_22/7(din6)
  pol1_in22_last_tap/2(sync_out) -> adder_1_22/1(sync)
  pol1_in22_last_tap/1(tap_out) -> adder_1_22/9(din8)
  pol1_in22_tap7/1(dout) -> pol1_in22_last_tap/1(din)
  pol1_in22_tap7/2(sync_out) -> pol1_in22_last_tap/2(sync)
  pol1_in22_tap7/3(coeff_out) -> pol1_in22_last_tap/3(coeff)
  pol1_in22_tap7/4(taps_out) -> adder_1_22/8(din7)
  pol1_in23_first_tap/1(dout) -> pol1_in23_tap2/1(din)
  pol1_in23_first_tap/2(sync_out) -> pol1_in23_tap2/2(sync)
  pol1_in23_first_tap/3(coeff_out) -> pol1_in23_tap2/3(coeff)
  pol1_in23_first_tap/4(taps_out) -> adder_1_23/2(din1)
  pol1_in23_tap2/1(dout) -> pol1_in23_tap3/1(din)
  pol1_in23_tap2/2(sync_out) -> pol1_in23_tap3/2(sync)
  pol1_in23_tap2/3(coeff_out) -> pol1_in23_tap3/3(coeff)
  pol1_in23_tap2/4(taps_out) -> adder_1_23/3(din2)
  pol1_in23_tap3/1(dout) -> pol1_in23_tap4/1(din)
  pol1_in23_tap3/2(sync_out) -> pol1_in23_tap4/2(sync)
  pol1_in23_tap3/3(coeff_out) -> pol1_in23_tap4/3(coeff)
  pol1_in23_tap3/4(taps_out) -> adder_1_23/4(din3)
  pol1_in23_tap4/1(dout) -> pol1_in23_tap5/1(din)
  pol1_in23_tap4/2(sync_out) -> pol1_in23_tap5/2(sync)
  pol1_in23_tap4/3(coeff_out) -> pol1_in23_tap5/3(coeff)
  pol1_in23_tap4/4(taps_out) -> adder_1_23/5(din4)
  pol1_in23_tap5/1(dout) -> pol1_in23_tap6/1(din)
  pol1_in23_tap5/2(sync_out) -> pol1_in23_tap6/2(sync)
  pol1_in23_tap5/3(coeff_out) -> pol1_in23_tap6/3(coeff)
  pol1_in23_tap5/4(taps_out) -> adder_1_23/6(din5)
  pol1_in23_tap6/1(dout) -> pol1_in23_tap7/1(din)
  pol1_in23_tap6/2(sync_out) -> pol1_in23_tap7/2(sync)
  pol1_in23_tap6/3(coeff_out) -> pol1_in23_tap7/3(coeff)
  pol1_in23_tap6/4(taps_out) -> adder_1_23/7(din6)
  pol1_in23_last_tap/2(sync_out) -> adder_1_23/1(sync)
  pol1_in23_last_tap/1(tap_out) -> adder_1_23/9(din8)
  pol1_in23_tap7/1(dout) -> pol1_in23_last_tap/1(din)
  pol1_in23_tap7/2(sync_out) -> pol1_in23_last_tap/2(sync)
  pol1_in23_tap7/3(coeff_out) -> pol1_in23_last_tap/3(coeff)
  pol1_in23_tap7/4(taps_out) -> adder_1_23/8(din7)
  pol1_in24_first_tap/1(dout) -> pol1_in24_tap2/1(din)
  pol1_in24_first_tap/2(sync_out) -> pol1_in24_tap2/2(sync)
  pol1_in24_first_tap/3(coeff_out) -> pol1_in24_tap2/3(coeff)
  pol1_in24_first_tap/4(taps_out) -> adder_1_24/2(din1)
  pol1_in24_tap2/1(dout) -> pol1_in24_tap3/1(din)
  pol1_in24_tap2/2(sync_out) -> pol1_in24_tap3/2(sync)
  pol1_in24_tap2/3(coeff_out) -> pol1_in24_tap3/3(coeff)
  pol1_in24_tap2/4(taps_out) -> adder_1_24/3(din2)
  pol1_in24_tap3/1(dout) -> pol1_in24_tap4/1(din)
  pol1_in24_tap3/2(sync_out) -> pol1_in24_tap4/2(sync)
  pol1_in24_tap3/3(coeff_out) -> pol1_in24_tap4/3(coeff)
  pol1_in24_tap3/4(taps_out) -> adder_1_24/4(din3)
  pol1_in24_tap4/1(dout) -> pol1_in24_tap5/1(din)
  pol1_in24_tap4/2(sync_out) -> pol1_in24_tap5/2(sync)
  pol1_in24_tap4/3(coeff_out) -> pol1_in24_tap5/3(coeff)
  pol1_in24_tap4/4(taps_out) -> adder_1_24/5(din4)
  pol1_in24_tap5/1(dout) -> pol1_in24_tap6/1(din)
  pol1_in24_tap5/2(sync_out) -> pol1_in24_tap6/2(sync)
  pol1_in24_tap5/3(coeff_out) -> pol1_in24_tap6/3(coeff)
  pol1_in24_tap5/4(taps_out) -> adder_1_24/6(din5)
  pol1_in24_tap6/1(dout) -> pol1_in24_tap7/1(din)
  pol1_in24_tap6/2(sync_out) -> pol1_in24_tap7/2(sync)
  pol1_in24_tap6/3(coeff_out) -> pol1_in24_tap7/3(coeff)
  pol1_in24_tap6/4(taps_out) -> adder_1_24/7(din6)
  pol1_in24_last_tap/2(sync_out) -> adder_1_24/1(sync)
  pol1_in24_last_tap/1(tap_out) -> adder_1_24/9(din8)
  pol1_in24_tap7/1(dout) -> pol1_in24_last_tap/1(din)
  pol1_in24_tap7/2(sync_out) -> pol1_in24_last_tap/2(sync)
  pol1_in24_tap7/3(coeff_out) -> pol1_in24_last_tap/3(coeff)
  pol1_in24_tap7/4(taps_out) -> adder_1_24/8(din7)
  pol1_in25_first_tap/1(dout) -> pol1_in25_tap2/1(din)
  pol1_in25_first_tap/2(sync_out) -> pol1_in25_tap2/2(sync)
  pol1_in25_first_tap/3(coeff_out) -> pol1_in25_tap2/3(coeff)
  pol1_in25_first_tap/4(taps_out) -> adder_1_25/2(din1)
  pol1_in25_tap2/1(dout) -> pol1_in25_tap3/1(din)
  pol1_in25_tap2/2(sync_out) -> pol1_in25_tap3/2(sync)
  pol1_in25_tap2/3(coeff_out) -> pol1_in25_tap3/3(coeff)
  pol1_in25_tap2/4(taps_out) -> adder_1_25/3(din2)
  pol1_in25_tap3/1(dout) -> pol1_in25_tap4/1(din)
  pol1_in25_tap3/2(sync_out) -> pol1_in25_tap4/2(sync)
  pol1_in25_tap3/3(coeff_out) -> pol1_in25_tap4/3(coeff)
  pol1_in25_tap3/4(taps_out) -> adder_1_25/4(din3)
  pol1_in25_tap4/1(dout) -> pol1_in25_tap5/1(din)
  pol1_in25_tap4/2(sync_out) -> pol1_in25_tap5/2(sync)
  pol1_in25_tap4/3(coeff_out) -> pol1_in25_tap5/3(coeff)
  pol1_in25_tap4/4(taps_out) -> adder_1_25/5(din4)
  pol1_in25_tap5/1(dout) -> pol1_in25_tap6/1(din)
  pol1_in25_tap5/2(sync_out) -> pol1_in25_tap6/2(sync)
  pol1_in25_tap5/3(coeff_out) -> pol1_in25_tap6/3(coeff)
  pol1_in25_tap5/4(taps_out) -> adder_1_25/6(din5)
  pol1_in25_tap6/1(dout) -> pol1_in25_tap7/1(din)
  pol1_in25_tap6/2(sync_out) -> pol1_in25_tap7/2(sync)
  pol1_in25_tap6/3(coeff_out) -> pol1_in25_tap7/3(coeff)
  pol1_in25_tap6/4(taps_out) -> adder_1_25/7(din6)
  pol1_in25_last_tap/2(sync_out) -> adder_1_25/1(sync)
  pol1_in25_last_tap/1(tap_out) -> adder_1_25/9(din8)
  pol1_in25_tap7/1(dout) -> pol1_in25_last_tap/1(din)
  pol1_in25_tap7/2(sync_out) -> pol1_in25_last_tap/2(sync)
  pol1_in25_tap7/3(coeff_out) -> pol1_in25_last_tap/3(coeff)
  pol1_in25_tap7/4(taps_out) -> adder_1_25/8(din7)
  pol1_in26_first_tap/1(dout) -> pol1_in26_tap2/1(din)
  pol1_in26_first_tap/2(sync_out) -> pol1_in26_tap2/2(sync)
  pol1_in26_first_tap/3(coeff_out) -> pol1_in26_tap2/3(coeff)
  pol1_in26_first_tap/4(taps_out) -> adder_1_26/2(din1)
  pol1_in26_tap2/1(dout) -> pol1_in26_tap3/1(din)
  pol1_in26_tap2/2(sync_out) -> pol1_in26_tap3/2(sync)
  pol1_in26_tap2/3(coeff_out) -> pol1_in26_tap3/3(coeff)
  pol1_in26_tap2/4(taps_out) -> adder_1_26/3(din2)
  pol1_in26_tap3/1(dout) -> pol1_in26_tap4/1(din)
  pol1_in26_tap3/2(sync_out) -> pol1_in26_tap4/2(sync)
  pol1_in26_tap3/3(coeff_out) -> pol1_in26_tap4/3(coeff)
  pol1_in26_tap3/4(taps_out) -> adder_1_26/4(din3)
  pol1_in26_tap4/1(dout) -> pol1_in26_tap5/1(din)
  pol1_in26_tap4/2(sync_out) -> pol1_in26_tap5/2(sync)
  pol1_in26_tap4/3(coeff_out) -> pol1_in26_tap5/3(coeff)
  pol1_in26_tap4/4(taps_out) -> adder_1_26/5(din4)
  pol1_in26_tap5/1(dout) -> pol1_in26_tap6/1(din)
  pol1_in26_tap5/2(sync_out) -> pol1_in26_tap6/2(sync)
  pol1_in26_tap5/3(coeff_out) -> pol1_in26_tap6/3(coeff)
  pol1_in26_tap5/4(taps_out) -> adder_1_26/6(din5)
  pol1_in26_tap6/1(dout) -> pol1_in26_tap7/1(din)
  pol1_in26_tap6/2(sync_out) -> pol1_in26_tap7/2(sync)
  pol1_in26_tap6/3(coeff_out) -> pol1_in26_tap7/3(coeff)
  pol1_in26_tap6/4(taps_out) -> adder_1_26/7(din6)
  pol1_in26_last_tap/2(sync_out) -> adder_1_26/1(sync)
  pol1_in26_last_tap/1(tap_out) -> adder_1_26/9(din8)
  pol1_in26_tap7/1(dout) -> pol1_in26_last_tap/1(din)
  pol1_in26_tap7/2(sync_out) -> pol1_in26_last_tap/2(sync)
  pol1_in26_tap7/3(coeff_out) -> pol1_in26_last_tap/3(coeff)
  pol1_in26_tap7/4(taps_out) -> adder_1_26/8(din7)
  pol1_in27_first_tap/1(dout) -> pol1_in27_tap2/1(din)
  pol1_in27_first_tap/2(sync_out) -> pol1_in27_tap2/2(sync)
  pol1_in27_first_tap/3(coeff_out) -> pol1_in27_tap2/3(coeff)
  pol1_in27_first_tap/4(taps_out) -> adder_1_27/2(din1)
  pol1_in27_tap2/1(dout) -> pol1_in27_tap3/1(din)
  pol1_in27_tap2/2(sync_out) -> pol1_in27_tap3/2(sync)
  pol1_in27_tap2/3(coeff_out) -> pol1_in27_tap3/3(coeff)
  pol1_in27_tap2/4(taps_out) -> adder_1_27/3(din2)
  pol1_in27_tap3/1(dout) -> pol1_in27_tap4/1(din)
  pol1_in27_tap3/2(sync_out) -> pol1_in27_tap4/2(sync)
  pol1_in27_tap3/3(coeff_out) -> pol1_in27_tap4/3(coeff)
  pol1_in27_tap3/4(taps_out) -> adder_1_27/4(din3)
  pol1_in27_tap4/1(dout) -> pol1_in27_tap5/1(din)
  pol1_in27_tap4/2(sync_out) -> pol1_in27_tap5/2(sync)
  pol1_in27_tap4/3(coeff_out) -> pol1_in27_tap5/3(coeff)
  pol1_in27_tap4/4(taps_out) -> adder_1_27/5(din4)
  pol1_in27_tap5/1(dout) -> pol1_in27_tap6/1(din)
  pol1_in27_tap5/2(sync_out) -> pol1_in27_tap6/2(sync)
  pol1_in27_tap5/3(coeff_out) -> pol1_in27_tap6/3(coeff)
  pol1_in27_tap5/4(taps_out) -> adder_1_27/6(din5)
  pol1_in27_tap6/1(dout) -> pol1_in27_tap7/1(din)
  pol1_in27_tap6/2(sync_out) -> pol1_in27_tap7/2(sync)
  pol1_in27_tap6/3(coeff_out) -> pol1_in27_tap7/3(coeff)
  pol1_in27_tap6/4(taps_out) -> adder_1_27/7(din6)
  pol1_in27_last_tap/2(sync_out) -> adder_1_27/1(sync)
  pol1_in27_last_tap/1(tap_out) -> adder_1_27/9(din8)
  pol1_in27_tap7/1(dout) -> pol1_in27_last_tap/1(din)
  pol1_in27_tap7/2(sync_out) -> pol1_in27_last_tap/2(sync)
  pol1_in27_tap7/3(coeff_out) -> pol1_in27_last_tap/3(coeff)
  pol1_in27_tap7/4(taps_out) -> adder_1_27/8(din7)
  pol1_in28_first_tap/1(dout) -> pol1_in28_tap2/1(din)
  pol1_in28_first_tap/2(sync_out) -> pol1_in28_tap2/2(sync)
  pol1_in28_first_tap/3(coeff_out) -> pol1_in28_tap2/3(coeff)
  pol1_in28_first_tap/4(taps_out) -> adder_1_28/2(din1)
  pol1_in28_tap2/1(dout) -> pol1_in28_tap3/1(din)
  pol1_in28_tap2/2(sync_out) -> pol1_in28_tap3/2(sync)
  pol1_in28_tap2/3(coeff_out) -> pol1_in28_tap3/3(coeff)
  pol1_in28_tap2/4(taps_out) -> adder_1_28/3(din2)
  pol1_in28_tap3/1(dout) -> pol1_in28_tap4/1(din)
  pol1_in28_tap3/2(sync_out) -> pol1_in28_tap4/2(sync)
  pol1_in28_tap3/3(coeff_out) -> pol1_in28_tap4/3(coeff)
  pol1_in28_tap3/4(taps_out) -> adder_1_28/4(din3)
  pol1_in28_tap4/1(dout) -> pol1_in28_tap5/1(din)
  pol1_in28_tap4/2(sync_out) -> pol1_in28_tap5/2(sync)
  pol1_in28_tap4/3(coeff_out) -> pol1_in28_tap5/3(coeff)
  pol1_in28_tap4/4(taps_out) -> adder_1_28/5(din4)
  pol1_in28_tap5/1(dout) -> pol1_in28_tap6/1(din)
  pol1_in28_tap5/2(sync_out) -> pol1_in28_tap6/2(sync)
  pol1_in28_tap5/3(coeff_out) -> pol1_in28_tap6/3(coeff)
  pol1_in28_tap5/4(taps_out) -> adder_1_28/6(din5)
  pol1_in28_tap6/1(dout) -> pol1_in28_tap7/1(din)
  pol1_in28_tap6/2(sync_out) -> pol1_in28_tap7/2(sync)
  pol1_in28_tap6/3(coeff_out) -> pol1_in28_tap7/3(coeff)
  pol1_in28_tap6/4(taps_out) -> adder_1_28/7(din6)
  pol1_in28_last_tap/2(sync_out) -> adder_1_28/1(sync)
  pol1_in28_last_tap/1(tap_out) -> adder_1_28/9(din8)
  pol1_in28_tap7/1(dout) -> pol1_in28_last_tap/1(din)
  pol1_in28_tap7/2(sync_out) -> pol1_in28_last_tap/2(sync)
  pol1_in28_tap7/3(coeff_out) -> pol1_in28_last_tap/3(coeff)
  pol1_in28_tap7/4(taps_out) -> adder_1_28/8(din7)
  pol1_in29_first_tap/1(dout) -> pol1_in29_tap2/1(din)
  pol1_in29_first_tap/2(sync_out) -> pol1_in29_tap2/2(sync)
  pol1_in29_first_tap/3(coeff_out) -> pol1_in29_tap2/3(coeff)
  pol1_in29_first_tap/4(taps_out) -> adder_1_29/2(din1)
  pol1_in29_tap2/1(dout) -> pol1_in29_tap3/1(din)
  pol1_in29_tap2/2(sync_out) -> pol1_in29_tap3/2(sync)
  pol1_in29_tap2/3(coeff_out) -> pol1_in29_tap3/3(coeff)
  pol1_in29_tap2/4(taps_out) -> adder_1_29/3(din2)
  pol1_in29_tap3/1(dout) -> pol1_in29_tap4/1(din)
  pol1_in29_tap3/2(sync_out) -> pol1_in29_tap4/2(sync)
  pol1_in29_tap3/3(coeff_out) -> pol1_in29_tap4/3(coeff)
  pol1_in29_tap3/4(taps_out) -> adder_1_29/4(din3)
  pol1_in29_tap4/1(dout) -> pol1_in29_tap5/1(din)
  pol1_in29_tap4/2(sync_out) -> pol1_in29_tap5/2(sync)
  pol1_in29_tap4/3(coeff_out) -> pol1_in29_tap5/3(coeff)
  pol1_in29_tap4/4(taps_out) -> adder_1_29/5(din4)
  pol1_in29_tap5/1(dout) -> pol1_in29_tap6/1(din)
  pol1_in29_tap5/2(sync_out) -> pol1_in29_tap6/2(sync)
  pol1_in29_tap5/3(coeff_out) -> pol1_in29_tap6/3(coeff)
  pol1_in29_tap5/4(taps_out) -> adder_1_29/6(din5)
  pol1_in29_tap6/1(dout) -> pol1_in29_tap7/1(din)
  pol1_in29_tap6/2(sync_out) -> pol1_in29_tap7/2(sync)
  pol1_in29_tap6/3(coeff_out) -> pol1_in29_tap7/3(coeff)
  pol1_in29_tap6/4(taps_out) -> adder_1_29/7(din6)
  pol1_in29_last_tap/2(sync_out) -> adder_1_29/1(sync)
  pol1_in29_last_tap/1(tap_out) -> adder_1_29/9(din8)
  pol1_in29_tap7/1(dout) -> pol1_in29_last_tap/1(din)
  pol1_in29_tap7/2(sync_out) -> pol1_in29_last_tap/2(sync)
  pol1_in29_tap7/3(coeff_out) -> pol1_in29_last_tap/3(coeff)
  pol1_in29_tap7/4(taps_out) -> adder_1_29/8(din7)
  pol1_in30_first_tap/1(dout) -> pol1_in30_tap2/1(din)
  pol1_in30_first_tap/2(sync_out) -> pol1_in30_tap2/2(sync)
  pol1_in30_first_tap/3(coeff_out) -> pol1_in30_tap2/3(coeff)
  pol1_in30_first_tap/4(taps_out) -> adder_1_30/2(din1)
  pol1_in30_tap2/1(dout) -> pol1_in30_tap3/1(din)
  pol1_in30_tap2/2(sync_out) -> pol1_in30_tap3/2(sync)
  pol1_in30_tap2/3(coeff_out) -> pol1_in30_tap3/3(coeff)
  pol1_in30_tap2/4(taps_out) -> adder_1_30/3(din2)
  pol1_in30_tap3/1(dout) -> pol1_in30_tap4/1(din)
  pol1_in30_tap3/2(sync_out) -> pol1_in30_tap4/2(sync)
  pol1_in30_tap3/3(coeff_out) -> pol1_in30_tap4/3(coeff)
  pol1_in30_tap3/4(taps_out) -> adder_1_30/4(din3)
  pol1_in30_tap4/1(dout) -> pol1_in30_tap5/1(din)
  pol1_in30_tap4/2(sync_out) -> pol1_in30_tap5/2(sync)
  pol1_in30_tap4/3(coeff_out) -> pol1_in30_tap5/3(coeff)
  pol1_in30_tap4/4(taps_out) -> adder_1_30/5(din4)
  pol1_in30_tap5/1(dout) -> pol1_in30_tap6/1(din)
  pol1_in30_tap5/2(sync_out) -> pol1_in30_tap6/2(sync)
  pol1_in30_tap5/3(coeff_out) -> pol1_in30_tap6/3(coeff)
  pol1_in30_tap5/4(taps_out) -> adder_1_30/6(din5)
  pol1_in30_tap6/1(dout) -> pol1_in30_tap7/1(din)
  pol1_in30_tap6/2(sync_out) -> pol1_in30_tap7/2(sync)
  pol1_in30_tap6/3(coeff_out) -> pol1_in30_tap7/3(coeff)
  pol1_in30_tap6/4(taps_out) -> adder_1_30/7(din6)
  pol1_in30_last_tap/2(sync_out) -> adder_1_30/1(sync)
  pol1_in30_last_tap/1(tap_out) -> adder_1_30/9(din8)
  pol1_in30_tap7/1(dout) -> pol1_in30_last_tap/1(din)
  pol1_in30_tap7/2(sync_out) -> pol1_in30_last_tap/2(sync)
  pol1_in30_tap7/3(coeff_out) -> pol1_in30_last_tap/3(coeff)
  pol1_in30_tap7/4(taps_out) -> adder_1_30/8(din7)
  pol1_in31_first_tap/1(dout) -> pol1_in31_tap2/1(din)
  pol1_in31_first_tap/2(sync_out) -> pol1_in31_tap2/2(sync)
  pol1_in31_first_tap/3(coeff_out) -> pol1_in31_tap2/3(coeff)
  pol1_in31_first_tap/4(taps_out) -> adder_1_31/2(din1)
  pol1_in31_tap2/1(dout) -> pol1_in31_tap3/1(din)
  pol1_in31_tap2/2(sync_out) -> pol1_in31_tap3/2(sync)
  pol1_in31_tap2/3(coeff_out) -> pol1_in31_tap3/3(coeff)
  pol1_in31_tap2/4(taps_out) -> adder_1_31/3(din2)
  pol1_in31_tap3/1(dout) -> pol1_in31_tap4/1(din)
  pol1_in31_tap3/2(sync_out) -> pol1_in31_tap4/2(sync)
  pol1_in31_tap3/3(coeff_out) -> pol1_in31_tap4/3(coeff)
  pol1_in31_tap3/4(taps_out) -> adder_1_31/4(din3)
  pol1_in31_tap4/1(dout) -> pol1_in31_tap5/1(din)
  pol1_in31_tap4/2(sync_out) -> pol1_in31_tap5/2(sync)
  pol1_in31_tap4/3(coeff_out) -> pol1_in31_tap5/3(coeff)
  pol1_in31_tap4/4(taps_out) -> adder_1_31/5(din4)
  pol1_in31_tap5/1(dout) -> pol1_in31_tap6/1(din)
  pol1_in31_tap5/2(sync_out) -> pol1_in31_tap6/2(sync)
  pol1_in31_tap5/3(coeff_out) -> pol1_in31_tap6/3(coeff)
  pol1_in31_tap5/4(taps_out) -> adder_1_31/6(din5)
  pol1_in31_tap6/1(dout) -> pol1_in31_tap7/1(din)
  pol1_in31_tap6/2(sync_out) -> pol1_in31_tap7/2(sync)
  pol1_in31_tap6/3(coeff_out) -> pol1_in31_tap7/3(coeff)
  pol1_in31_tap6/4(taps_out) -> adder_1_31/7(din6)
  pol1_in31_last_tap/2(sync_out) -> adder_1_31/1(sync)
  pol1_in31_last_tap/1(tap_out) -> adder_1_31/9(din8)
  pol1_in31_tap7/1(dout) -> pol1_in31_last_tap/1(din)
  pol1_in31_tap7/2(sync_out) -> pol1_in31_last_tap/2(sync)
  pol1_in31_tap7/3(coeff_out) -> pol1_in31_last_tap/3(coeff)
  pol1_in31_tap7/4(taps_out) -> adder_1_31/8(din7)
  pol1_in32_first_tap/1(dout) -> pol1_in32_tap2/1(din)
  pol1_in32_first_tap/2(sync_out) -> pol1_in32_tap2/2(sync)
  pol1_in32_first_tap/3(coeff_out) -> pol1_in32_tap2/3(coeff)
  pol1_in32_first_tap/4(taps_out) -> adder_1_32/2(din1)
  pol1_in32_tap2/1(dout) -> pol1_in32_tap3/1(din)
  pol1_in32_tap2/2(sync_out) -> pol1_in32_tap3/2(sync)
  pol1_in32_tap2/3(coeff_out) -> pol1_in32_tap3/3(coeff)
  pol1_in32_tap2/4(taps_out) -> adder_1_32/3(din2)
  pol1_in32_tap3/1(dout) -> pol1_in32_tap4/1(din)
  pol1_in32_tap3/2(sync_out) -> pol1_in32_tap4/2(sync)
  pol1_in32_tap3/3(coeff_out) -> pol1_in32_tap4/3(coeff)
  pol1_in32_tap3/4(taps_out) -> adder_1_32/4(din3)
  pol1_in32_tap4/1(dout) -> pol1_in32_tap5/1(din)
  pol1_in32_tap4/2(sync_out) -> pol1_in32_tap5/2(sync)
  pol1_in32_tap4/3(coeff_out) -> pol1_in32_tap5/3(coeff)
  pol1_in32_tap4/4(taps_out) -> adder_1_32/5(din4)
  pol1_in32_tap5/1(dout) -> pol1_in32_tap6/1(din)
  pol1_in32_tap5/2(sync_out) -> pol1_in32_tap6/2(sync)
  pol1_in32_tap5/3(coeff_out) -> pol1_in32_tap6/3(coeff)
  pol1_in32_tap5/4(taps_out) -> adder_1_32/6(din5)
  pol1_in32_tap6/1(dout) -> pol1_in32_tap7/1(din)
  pol1_in32_tap6/2(sync_out) -> pol1_in32_tap7/2(sync)
  pol1_in32_tap6/3(coeff_out) -> pol1_in32_tap7/3(coeff)
  pol1_in32_tap6/4(taps_out) -> adder_1_32/7(din6)
  pol1_in32_last_tap/2(sync_out) -> adder_1_32/1(sync)
  pol1_in32_last_tap/1(tap_out) -> adder_1_32/9(din8)
  pol1_in32_tap7/1(dout) -> pol1_in32_last_tap/1(din)
  pol1_in32_tap7/2(sync_out) -> pol1_in32_last_tap/2(sync)
  pol1_in32_tap7/3(coeff_out) -> pol1_in32_last_tap/3(coeff)
  pol1_in32_tap7/4(taps_out) -> adder_1_32/8(din7)
